simulink model "pokus07_video"  (R2023a)
settings: Solver=VariableStepAuto  StartTime=0.0  StopTime=10.0  RelTol=1e-3
undefined symbols (not defined in the file): c
libraries: Miscellaneous x840, Memory_Blocks_Lib x251, Decoders_Lib x10, simulink_extras x10, Counters_Lib x4, Bit_Multiplexers_Lib x1, Byte_Multiplexers_Lib x1
(part 2 of 5)

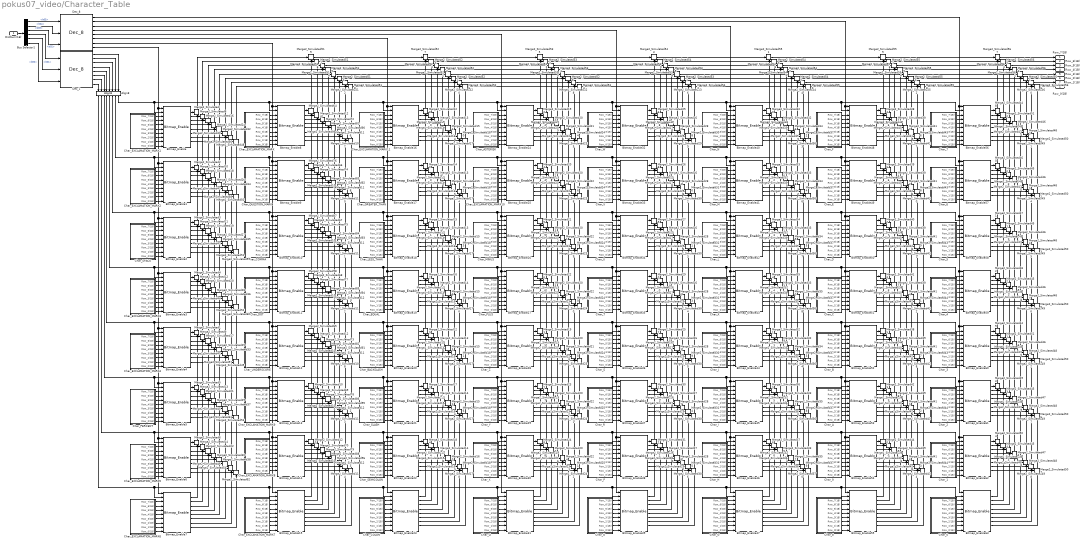
== system pokus07_video/Character_Table ==
  OrdNum(1B) : Inport
  Align8 : Miscellaneous/Align8  SystemSampleTime=-1  VariantActivationTime=update diagram  Latency=0  AutoFrameSizeCalculation=off
  Bitmap_Enable{,1..63} (64 alike) : Miscellaneous/Bitmap_Enable  SystemSampleTime=-1  VariantActivationTime=update diagram  Latency=0  AutoFrameSizeCalculation=off
  Bus Selector1 : BusSelector  OutputSignals=b05,b04,b03,b02,b01,b00
  Char_0 : Subsystem
  Char_1 : Subsystem
  Char_2 : Subsystem
  Char_3 : Subsystem
  Char_4 : Subsystem
  Char_5 : Subsystem
  Char_6 : Subsystem
  Char_7 : Subsystem
  Char_8 : Subsystem
  Char_9 : Subsystem
  Char_A : Subsystem
  Char_ASTERISK : Subsystem
  Char_B : Subsystem
  Char_BACKSLASH : Subsystem
  Char_C : Subsystem
  Char_COLON : Subsystem
  Char_COMMA : Subsystem
  Char_D : Subsystem
  Char_DOT : Subsystem
  Char_E : Subsystem
  Char_EQUAL : Subsystem
  Char_EXCLAMATION_MARK : Subsystem
  Char_EXCLAMATION_MARK1 : Subsystem
  Char_EXCLAMATION_MARK10 : Subsystem
  Char_EXCLAMATION_MARK11 : Subsystem
  Char_EXCLAMATION_MARK2 : Subsystem
  Char_EXCLAMATION_MARK3 : Subsystem
  Char_EXCLAMATION_MARK4 : Subsystem
  Char_EXCLAMATION_MARK5 : Subsystem
  Char_EXCLAMATION_MARK6 : Subsystem
  Char_EXCLAMATION_MARK7 : Subsystem
  Char_EXCLAMATION_MARK8 : Subsystem
  Char_EXCLAMATION_MARK9 : Subsystem
  Char_F : Subsystem
  Char_G : Subsystem
  Char_GREATER_THAN : Subsystem
  Char_H : Subsystem
  Char_I : Subsystem
  Char_J : Subsystem
  Char_K : Subsystem
  Char_L : Subsystem
  Char_LESS_THAN : Subsystem
  Char_M : Subsystem
  Char_MINUS : Subsystem
  Char_N : Subsystem
  Char_O : Subsystem
  Char_P : Subsystem
  Char_PERCENT : Subsystem
  Char_PLUS : Subsystem
  Char_Q : Subsystem
  Char_QUESTION_MARK : Subsystem
  Char_R : Subsystem
  Char_S : Subsystem
  Char_SEMICOLON : Subsystem
  Char_SLASH : Subsystem
  Char_SPACE : Subsystem
  Char_T : Subsystem
  Char_U : Subsystem
  Char_UNDERSCORE : Subsystem
  Char_V : Subsystem
  Char_W : Subsystem
  Char_X : Subsystem
  Char_Y : Subsystem
  Char_Z : Subsystem
  Dec_1 : Decoders_Lib/Dec_8  SystemSampleTime=-1  VariantActivationTime=update diagram  Latency=0  AutoFrameSizeCalculation=off
  Dec_8 : Decoders_Lib/Dec_8  SystemSampleTime=-1  VariantActivationTime=update diagram  Latency=0  AutoFrameSizeCalculation=off
  Merge2_Simulated{,1..6,8..14,16..22,24..30,32..38,40..46,48..54,56..62,64..70,72..79,81..88,90..96,98..105,107..114,116..123,126..134,136..143,145..152,154..160,162..169,171..178,180..187,190..198,200..207,209..216,218..224,226..233,235..242,244..251,254..262,264..271,273..280,282..288,290..297,299..306,308..315,318..326,328..335,337..344,346..352,354..361,363..370,372..379,382..390,392..399,401..408,410..416,418..425,427..434,436..443,446..454,456..463,465..472,474..480,482..489,491..498,500..507,510..567} (504 alike) : Miscellaneous/Merge2_Simulated  SystemSampleTime=-1  VariantActivationTime=update diagram  Latency=0  AutoFrameSizeCalculation=off
      settings: PortSchema="{\"entries\":[{\"content\":{\"sides\":[{\"content\":{\"connectorIds\":[\"In1\"]},\"type\":\"ConnectorPlacement.EquallySpacedRectSide\",\"uuid\":\"74758995-5ec8-49f8-a534-c3a678c5c312\"},{\"content\":{\"side\":\"RIGHT\"},\"type\":\"ConnectorPlacement.EquallySpacedRectSide\",\"uuid\":\"c467dbeb-9f00-48b9-a78d-a08162163a10\"},{\"content\":{\"connectorIds\":[\"Out1\"],\"side\":\"TOP\"},\"type\":\"ConnectorPlacement.EquallySpacedRectSide\",\"uuid\":\"39dea3b5-6733-4ade-ab22-e62d310be187\"},{\"content\":{\"connectorIds\":[\"In2\"],\"side\":\"BOTTOM\"},\"type\":\"ConnectorPlacement.EquallySpacedRectSide\",\"uuid\":\"73149fc1-24d9-4bdc-92e2-12fb1d742836\"}]},\"type\":\"ConnectorPlacement.EquallySpacedConnector\",\"uuid\":\"fd2226dc-a4d3-43ad-9cda-54babd09ac78\"}],\"packageUris\":[\"http://schema.mathworks.com/mf0/Connector/R2020b\"],\"version\":\"1.0\"}"
  Row_7(1B) : Outport
  Row_6(1B) : Outport  Port=2
  Row_5(1B) : Outport  Port=3
  Row_4(1B) : Outport  Port=4
  Row_3(1B) : Outport  Port=5
  Row_2(1B) : Outport  Port=6
  Row_1(1B) : Outport  Port=7
  Row_0(1B) : Outport  Port=8
  wires:
  Char_EXCLAMATION_MARK1/1(Row_7(1B)) -> Bitmap_Enable/3
  Char_EXCLAMATION_MARK1/2(Row_6(1B)) -> Bitmap_Enable/4
  Char_EXCLAMATION_MARK1/3(Row_5(1B)) -> Bitmap_Enable/5
  Char_EXCLAMATION_MARK1/4(Row_4(1B)) -> Bitmap_Enable/6
  Char_EXCLAMATION_MARK1/5(Row_3(1B)) -> Bitmap_Enable/7
  Char_EXCLAMATION_MARK1/6(Row_2(1B)) -> Bitmap_Enable/8
  Char_EXCLAMATION_MARK1/7(Row_1(1B)) -> Bitmap_Enable/9
  Char_EXCLAMATION_MARK1/8(Row_0(1B)) -> Bitmap_Enable/10
  Char_EXCLAMATION_MARK2/8(Row_0(1B)) -> Bitmap_Enable1/10
  Char_EXCLAMATION_MARK2/3(Row_5(1B)) -> Bitmap_Enable1/5
  Char_EXCLAMATION_MARK2/4(Row_4(1B)) -> Bitmap_Enable1/6
  Char_EXCLAMATION_MARK2/1(Row_7(1B)) -> Bitmap_Enable1/3
  Char_EXCLAMATION_MARK2/2(Row_6(1B)) -> Bitmap_Enable1/4
  Char_EXCLAMATION_MARK2/5(Row_3(1B)) -> Bitmap_Enable1/7
  Char_EXCLAMATION_MARK2/6(Row_2(1B)) -> Bitmap_Enable1/8
  Char_EXCLAMATION_MARK2/7(Row_1(1B)) -> Bitmap_Enable1/9
  Char_SPACE/8(Row_0(1B)) -> Bitmap_Enable2/10
  Char_SPACE/3(Row_5(1B)) -> Bitmap_Enable2/5
  Char_SPACE/4(Row_4(1B)) -> Bitmap_Enable2/6
  Char_SPACE/1(Row_7(1B)) -> Bitmap_Enable2/3
  Char_SPACE/2(Row_6(1B)) -> Bitmap_Enable2/4
  Char_SPACE/5(Row_3(1B)) -> Bitmap_Enable2/7
  Char_SPACE/6(Row_2(1B)) -> Bitmap_Enable2/8
  Char_SPACE/7(Row_1(1B)) -> Bitmap_Enable2/9
  Char_EXCLAMATION_MARK3/8(Row_0(1B)) -> Bitmap_Enable3/10
  Char_EXCLAMATION_MARK3/3(Row_5(1B)) -> Bitmap_Enable3/5
  Char_EXCLAMATION_MARK3/4(Row_4(1B)) -> Bitmap_Enable3/6
  Char_EXCLAMATION_MARK3/1(Row_7(1B)) -> Bitmap_Enable3/3
  Char_EXCLAMATION_MARK3/2(Row_6(1B)) -> Bitmap_Enable3/4
  Char_EXCLAMATION_MARK3/5(Row_3(1B)) -> Bitmap_Enable3/7
  Char_EXCLAMATION_MARK3/6(Row_2(1B)) -> Bitmap_Enable3/8
  Char_EXCLAMATION_MARK3/7(Row_1(1B)) -> Bitmap_Enable3/9
  Char_EXCLAMATION_MARK5/5(Row_3(1B)) -> Bitmap_Enable6/7
  Char_PERCENT/4(Row_4(1B)) -> Bitmap_Enable5/6
  Char_PERCENT/3(Row_5(1B)) -> Bitmap_Enable5/5
  Char_EXCLAMATION_MARK5/7(Row_1(1B)) -> Bitmap_Enable6/9
  Char_EXCLAMATION_MARK5/4(Row_4(1B)) -> Bitmap_Enable6/6
  Char_EXCLAMATION_MARK5/2(Row_6(1B)) -> Bitmap_Enable6/4
  Char_PERCENT/8(Row_0(1B)) -> Bitmap_Enable5/10
  Char_EXCLAMATION_MARK5/8(Row_0(1B)) -> Bitmap_Enable6/10
  Char_EXCLAMATION_MARK5/1(Row_7(1B)) -> Bitmap_Enable6/3
  Char_PERCENT/2(Row_6(1B)) -> Bitmap_Enable5/4
  Char_EXCLAMATION_MARK5/3(Row_5(1B)) -> Bitmap_Enable6/5
  Char_EXCLAMATION_MARK6/7(Row_1(1B)) -> Bitmap_Enable7/9
  Char_PERCENT/6(Row_2(1B)) -> Bitmap_Enable5/8
  Char_PERCENT/1(Row_7(1B)) -> Bitmap_Enable5/3
  Char_EXCLAMATION_MARK6/8(Row_0(1B)) -> Bitmap_Enable7/10
  Char_EXCLAMATION_MARK6/6(Row_2(1B)) -> Bitmap_Enable7/8
  Char_EXCLAMATION_MARK6/4(Row_4(1B)) -> Bitmap_Enable7/6
  Char_EXCLAMATION_MARK6/3(Row_5(1B)) -> Bitmap_Enable7/5
  Char_EXCLAMATION_MARK4/8(Row_0(1B)) -> Bitmap_Enable4/10
  Char_EXCLAMATION_MARK4/3(Row_5(1B)) -> Bitmap_Enable4/5
  Char_EXCLAMATION_MARK4/4(Row_4(1B)) -> Bitmap_Enable4/6
  Char_PERCENT/7(Row_1(1B)) -> Bitmap_Enable5/9
  Char_EXCLAMATION_MARK5/6(Row_2(1B)) -> Bitmap_Enable6/8
  Char_EXCLAMATION_MARK4/1(Row_7(1B)) -> Bitmap_Enable4/3
  Char_EXCLAMATION_MARK4/2(Row_6(1B)) -> Bitmap_Enable4/4
  Char_EXCLAMATION_MARK6/2(Row_6(1B)) -> Bitmap_Enable7/4
  Char_EXCLAMATION_MARK4/5(Row_3(1B)) -> Bitmap_Enable4/7
  Char_EXCLAMATION_MARK6/1(Row_7(1B)) -> Bitmap_Enable7/3
  Char_EXCLAMATION_MARK6/5(Row_3(1B)) -> Bitmap_Enable7/7
  Char_EXCLAMATION_MARK4/6(Row_2(1B)) -> Bitmap_Enable4/8
  Char_EXCLAMATION_MARK4/7(Row_1(1B)) -> Bitmap_Enable4/9
  Char_PERCENT/5(Row_3(1B)) -> Bitmap_Enable5/7
  Char_COMMA/5(Row_3(1B)) -> Bitmap_Enable10/7
  Char_QUESTION_MARK/4(Row_4(1B)) -> Bitmap_Enable9/6
  Char_QUESTION_MARK/3(Row_5(1B)) -> Bitmap_Enable9/5
  Char_COMMA/7(Row_1(1B)) -> Bitmap_Enable10/9
  Char_COMMA/4(Row_4(1B)) -> Bitmap_Enable10/6
  Char_COMMA/2(Row_6(1B)) -> Bitmap_Enable10/4
  Char_COMMA/1(Row_7(1B)) -> Bitmap_Enable10/3
  Char_QUESTION_MARK/2(Row_6(1B)) -> Bitmap_Enable9/4
  Char_COMMA/3(Row_5(1B)) -> Bitmap_Enable10/5
  Char_DOT/8(Row_0(1B)) -> Bitmap_Enable11/10
  Char_DOT/6(Row_2(1B)) -> Bitmap_Enable11/8
  Char_EXCLAMATION_MARK9/1(Row_7(1B)) -> Bitmap_Enable13/3
  Char_UNDERSCORE/1(Row_7(1B)) -> Bitmap_Enable12/3
  Char_EXCLAMATION_MARK9/2(Row_6(1B)) -> Bitmap_Enable13/4
  Char_EXCLAMATION_MARK8/3(Row_5(1B)) -> Bitmap_Enable14/4
  Char_EXCLAMATION_MARK9/4(Row_4(1B)) -> Bitmap_Enable13/6
  Char_EXCLAMATION_MARK8/8(Row_0(1B)) -> Bitmap_Enable14/9
  Char_EXCLAMATION_MARK8/7(Row_1(1B)) -> Bitmap_Enable14/8
  Char_EXCLAMATION_MARK8/5(Row_3(1B)) -> Bitmap_Enable14/6
  Char_EXCLAMATION_MARK7/8(Row_0(1B)) -> Bitmap_Enable15/10
  Char_UNDERSCORE/8(Row_0(1B)) -> Bitmap_Enable12/10
  Char_EXCLAMATION_MARK7/1(Row_7(1B)) -> Bitmap_Enable15/3
  Char_EXCLAMATION_MARK7/6(Row_2(1B)) -> Bitmap_Enable15/8
  Char_DOT/7(Row_1(1B)) -> Bitmap_Enable11/9
  Char_QUESTION_MARK/6(Row_2(1B)) -> Bitmap_Enable9/8
  Char_QUESTION_MARK/1(Row_7(1B)) -> Bitmap_Enable9/3
  Char_EXCLAMATION_MARK8/6(Row_2(1B)) -> Bitmap_Enable14/7
  Char_UNDERSCORE/5(Row_3(1B)) -> Bitmap_Enable12/7
  Char_EXCLAMATION_MARK9/5(Row_3(1B)) -> Bitmap_Enable13/7
  Char_UNDERSCORE/3(Row_5(1B)) -> Bitmap_Enable12/5
  Char_EXCLAMATION_MARK7/5(Row_3(1B)) -> Bitmap_Enable15/7
  ? -> Bitmap_Enable14/10
  Char_DOT/4(Row_4(1B)) -> Bitmap_Enable11/6
  Char_EXCLAMATION_MARK7/3(Row_5(1B)) -> Bitmap_Enable15/5
  Char_DOT/3(Row_5(1B)) -> Bitmap_Enable11/5
  Char_EXCLAMATION_MARK7/2(Row_6(1B)) -> Bitmap_Enable15/4
  Char_QUESTION_MARK/8(Row_0(1B)) -> Bitmap_Enable9/10
  Char_COMMA/8(Row_0(1B)) -> Bitmap_Enable10/10
  Char_EXCLAMATION_MARK7/4(Row_4(1B)) -> Bitmap_Enable15/6
  Char_UNDERSCORE/6(Row_2(1B)) -> Bitmap_Enable12/8
  Char_UNDERSCORE/7(Row_1(1B)) -> Bitmap_Enable12/9
  Char_UNDERSCORE/4(Row_4(1B)) -> Bitmap_Enable12/6
  Char_UNDERSCORE/2(Row_6(1B)) -> Bitmap_Enable12/4
  Char_EXCLAMATION_MARK8/2(Row_6(1B)) -> Bitmap_Enable14/3
  Char_EXCLAMATION_MARK9/8(Row_0(1B)) -> Bitmap_Enable13/10
  Char_EXCLAMATION_MARK9/6(Row_2(1B)) -> Bitmap_Enable13/8
  Char_EXCLAMATION_MARK9/7(Row_1(1B)) -> Bitmap_Enable13/9
  Char_EXCLAMATION_MARK9/3(Row_5(1B)) -> Bitmap_Enable13/5
  Char_EXCLAMATION_MARK/8(Row_0(1B)) -> Bitmap_Enable8/10
  Char_EXCLAMATION_MARK/3(Row_5(1B)) -> Bitmap_Enable8/5
  Char_EXCLAMATION_MARK7/7(Row_1(1B)) -> Bitmap_Enable15/9
  Char_EXCLAMATION_MARK/4(Row_4(1B)) -> Bitmap_Enable8/6
  Char_QUESTION_MARK/7(Row_1(1B)) -> Bitmap_Enable9/9
  Char_COMMA/6(Row_2(1B)) -> Bitmap_Enable10/8
  Char_EXCLAMATION_MARK/1(Row_7(1B)) -> Bitmap_Enable8/3
  Char_EXCLAMATION_MARK/2(Row_6(1B)) -> Bitmap_Enable8/4
  Char_DOT/2(Row_6(1B)) -> Bitmap_Enable11/4
  Char_EXCLAMATION_MARK/5(Row_3(1B)) -> Bitmap_Enable8/7
  Char_DOT/1(Row_7(1B)) -> Bitmap_Enable11/3
  Char_DOT/5(Row_3(1B)) -> Bitmap_Enable11/7
  Char_EXCLAMATION_MARK/6(Row_2(1B)) -> Bitmap_Enable8/8
  Char_EXCLAMATION_MARK/7(Row_1(1B)) -> Bitmap_Enable8/9
  Char_EXCLAMATION_MARK8/4(Row_4(1B)) -> Bitmap_Enable14/5
  Char_QUESTION_MARK/5(Row_3(1B)) -> Bitmap_Enable9/7
  Char_LESS_THAN/5(Row_3(1B)) -> Bitmap_Enable18/7
  Char_GREATER_THAN/4(Row_4(1B)) -> Bitmap_Enable17/6
  Char_GREATER_THAN/3(Row_5(1B)) -> Bitmap_Enable17/5
  Char_LESS_THAN/7(Row_1(1B)) -> Bitmap_Enable18/9
  Char_LESS_THAN/4(Row_4(1B)) -> Bitmap_Enable18/6
  Char_LESS_THAN/2(Row_6(1B)) -> Bitmap_Enable18/4
  Char_LESS_THAN/1(Row_7(1B)) -> Bitmap_Enable18/3
  Char_GREATER_THAN/2(Row_6(1B)) -> Bitmap_Enable17/4
  Char_LESS_THAN/3(Row_5(1B)) -> Bitmap_Enable18/5
  Char_EQUAL/8(Row_0(1B)) -> Bitmap_Enable19/10
  Char_EQUAL/6(Row_2(1B)) -> Bitmap_Enable19/8
  Char_SLASH/1(Row_7(1B)) -> Bitmap_Enable21/3
  Char_BACKSLASH/1(Row_7(1B)) -> Bitmap_Enable20/3
  Char_SLASH/2(Row_6(1B)) -> Bitmap_Enable21/4
  Char_SEMICOLON/2(Row_6(1B)) -> Bitmap_Enable22/4
  Char_SLASH/4(Row_4(1B)) -> Bitmap_Enable21/6
  Char_SEMICOLON/7(Row_1(1B)) -> Bitmap_Enable22/9
  Char_SEMICOLON/6(Row_2(1B)) -> Bitmap_Enable22/8
  Char_SEMICOLON/4(Row_4(1B)) -> Bitmap_Enable22/6
  Char_COLON/8(Row_0(1B)) -> Bitmap_Enable23/10
  Char_BACKSLASH/8(Row_0(1B)) -> Bitmap_Enable20/10
  Char_COLON/1(Row_7(1B)) -> Bitmap_Enable23/3
  Char_COLON/6(Row_2(1B)) -> Bitmap_Enable23/8
  Char_EQUAL/7(Row_1(1B)) -> Bitmap_Enable19/9
  Char_GREATER_THAN/6(Row_2(1B)) -> Bitmap_Enable17/8
  Char_GREATER_THAN/1(Row_7(1B)) -> Bitmap_Enable17/3
  Char_SEMICOLON/5(Row_3(1B)) -> Bitmap_Enable22/7
  Char_BACKSLASH/5(Row_3(1B)) -> Bitmap_Enable20/7
  Char_SLASH/5(Row_3(1B)) -> Bitmap_Enable21/7
  Char_BACKSLASH/3(Row_5(1B)) -> Bitmap_Enable20/5
  Char_COLON/5(Row_3(1B)) -> Bitmap_Enable23/7
  Char_SEMICOLON/8(Row_0(1B)) -> Bitmap_Enable22/10
  Char_EQUAL/4(Row_4(1B)) -> Bitmap_Enable19/6
  Char_COLON/3(Row_5(1B)) -> Bitmap_Enable23/5
  Char_EQUAL/3(Row_5(1B)) -> Bitmap_Enable19/5
  Char_COLON/2(Row_6(1B)) -> Bitmap_Enable23/4
  Char_GREATER_THAN/8(Row_0(1B)) -> Bitmap_Enable17/10
  Char_LESS_THAN/8(Row_0(1B)) -> Bitmap_Enable18/10
  Char_COLON/4(Row_4(1B)) -> Bitmap_Enable23/6
  Char_BACKSLASH/6(Row_2(1B)) -> Bitmap_Enable20/8
  Char_BACKSLASH/7(Row_1(1B)) -> Bitmap_Enable20/9
  Char_BACKSLASH/4(Row_4(1B)) -> Bitmap_Enable20/6
  Char_BACKSLASH/2(Row_6(1B)) -> Bitmap_Enable20/4
  Char_SEMICOLON/1(Row_7(1B)) -> Bitmap_Enable22/3
  Char_SLASH/8(Row_0(1B)) -> Bitmap_Enable21/10
  Char_SLASH/6(Row_2(1B)) -> Bitmap_Enable21/8
  Char_SLASH/7(Row_1(1B)) -> Bitmap_Enable21/9
  Char_SLASH/3(Row_5(1B)) -> Bitmap_Enable21/5
  Char_EXCLAMATION_MARK11/8(Row_0(1B)) -> Bitmap_Enable16/10
  Char_EXCLAMATION_MARK11/3(Row_5(1B)) -> Bitmap_Enable16/5
  Char_COLON/7(Row_1(1B)) -> Bitmap_Enable23/9
  Char_EXCLAMATION_MARK11/4(Row_4(1B)) -> Bitmap_Enable16/6
  Char_GREATER_THAN/7(Row_1(1B)) -> Bitmap_Enable17/9
  Char_LESS_THAN/6(Row_2(1B)) -> Bitmap_Enable18/8
  Char_EXCLAMATION_MARK11/1(Row_7(1B)) -> Bitmap_Enable16/3
  Char_EXCLAMATION_MARK11/2(Row_6(1B)) -> Bitmap_Enable16/4
  Char_EQUAL/2(Row_6(1B)) -> Bitmap_Enable19/4
  Char_EXCLAMATION_MARK11/5(Row_3(1B)) -> Bitmap_Enable16/7
  Char_EQUAL/1(Row_7(1B)) -> Bitmap_Enable19/3
  Char_EQUAL/5(Row_3(1B)) -> Bitmap_Enable19/7
  Char_EXCLAMATION_MARK11/6(Row_2(1B)) -> Bitmap_Enable16/8
  Char_EXCLAMATION_MARK11/7(Row_1(1B)) -> Bitmap_Enable16/9
  Char_SEMICOLON/3(Row_5(1B)) -> Bitmap_Enable22/5
  Char_GREATER_THAN/5(Row_3(1B)) -> Bitmap_Enable17/7
  Char_MINUS/5(Row_3(1B)) -> Bitmap_Enable26/7
  Char_EXCLAMATION_MARK10/4(Row_4(1B)) -> Bitmap_Enable25/6
  Char_EXCLAMATION_MARK10/3(Row_5(1B)) -> Bitmap_Enable25/5
  Char_MINUS/7(Row_1(1B)) -> Bitmap_Enable26/9
  Char_MINUS/4(Row_4(1B)) -> Bitmap_Enable26/6
  Char_MINUS/2(Row_6(1B)) -> Bitmap_Enable26/4
  Char_MINUS/1(Row_7(1B)) -> Bitmap_Enable26/3
  Char_EXCLAMATION_MARK10/2(Row_6(1B)) -> Bitmap_Enable25/4
  Char_MINUS/3(Row_5(1B)) -> Bitmap_Enable26/5
  Char_PLUS/8(Row_0(1B)) -> Bitmap_Enable27/10
  Char_PLUS/6(Row_2(1B)) -> Bitmap_Enable27/8
  Char_Y/1(Row_7(1B)) -> Bitmap_Enable29/3
  Char_Z/1(Row_7(1B)) -> Bitmap_Enable28/3
  Char_Y/2(Row_6(1B)) -> Bitmap_Enable29/4
  Char_X/2(Row_6(1B)) -> Bitmap_Enable30/4
  Char_Y/4(Row_4(1B)) -> Bitmap_Enable29/6
  Char_X/7(Row_1(1B)) -> Bitmap_Enable30/9
  Char_X/6(Row_2(1B)) -> Bitmap_Enable30/8
  Char_X/4(Row_4(1B)) -> Bitmap_Enable30/6
  Char_Q/8(Row_0(1B)) -> Bitmap_Enable31/10
  Char_Z/8(Row_0(1B)) -> Bitmap_Enable28/10
  Char_Q/1(Row_7(1B)) -> Bitmap_Enable31/3
  Char_Q/6(Row_2(1B)) -> Bitmap_Enable31/8
  Char_PLUS/7(Row_1(1B)) -> Bitmap_Enable27/9
  Char_EXCLAMATION_MARK10/6(Row_2(1B)) -> Bitmap_Enable25/8
  Char_EXCLAMATION_MARK10/1(Row_7(1B)) -> Bitmap_Enable25/3
  Char_X/5(Row_3(1B)) -> Bitmap_Enable30/7
  Char_Z/5(Row_3(1B)) -> Bitmap_Enable28/7
  Char_Y/5(Row_3(1B)) -> Bitmap_Enable29/7
  Char_Z/3(Row_5(1B)) -> Bitmap_Enable28/5
  Char_Q/5(Row_3(1B)) -> Bitmap_Enable31/7
  Char_X/8(Row_0(1B)) -> Bitmap_Enable30/10
  Char_PLUS/4(Row_4(1B)) -> Bitmap_Enable27/6
  Char_Q/3(Row_5(1B)) -> Bitmap_Enable31/5
  Char_PLUS/3(Row_5(1B)) -> Bitmap_Enable27/5
  Char_Q/2(Row_6(1B)) -> Bitmap_Enable31/4
  Char_EXCLAMATION_MARK10/8(Row_0(1B)) -> Bitmap_Enable25/10
  Char_MINUS/8(Row_0(1B)) -> Bitmap_Enable26/10
  Char_Q/4(Row_4(1B)) -> Bitmap_Enable31/6
  Char_Z/6(Row_2(1B)) -> Bitmap_Enable28/8
  Char_Z/7(Row_1(1B)) -> Bitmap_Enable28/9
  Char_Z/4(Row_4(1B)) -> Bitmap_Enable28/6
  Char_Z/2(Row_6(1B)) -> Bitmap_Enable28/4
  Char_X/1(Row_7(1B)) -> Bitmap_Enable30/3
  Char_Y/8(Row_0(1B)) -> Bitmap_Enable29/10
  Char_Y/6(Row_2(1B)) -> Bitmap_Enable29/8
  Char_Y/7(Row_1(1B)) -> Bitmap_Enable29/9
  Char_Y/3(Row_5(1B)) -> Bitmap_Enable29/5
  Char_ASTERISK/8(Row_0(1B)) -> Bitmap_Enable24/10
  Char_ASTERISK/3(Row_5(1B)) -> Bitmap_Enable24/5
  Char_Q/7(Row_1(1B)) -> Bitmap_Enable31/9
  Char_ASTERISK/4(Row_4(1B)) -> Bitmap_Enable24/6
  Char_EXCLAMATION_MARK10/7(Row_1(1B)) -> Bitmap_Enable25/9
  Char_MINUS/6(Row_2(1B)) -> Bitmap_Enable26/8
  Char_ASTERISK/1(Row_7(1B)) -> Bitmap_Enable24/3
  Char_ASTERISK/2(Row_6(1B)) -> Bitmap_Enable24/4
  Char_PLUS/2(Row_6(1B)) -> Bitmap_Enable27/4
  Char_ASTERISK/5(Row_3(1B)) -> Bitmap_Enable24/7
  Char_PLUS/1(Row_7(1B)) -> Bitmap_Enable27/3
  Char_PLUS/5(Row_3(1B)) -> Bitmap_Enable27/7
  Char_ASTERISK/6(Row_2(1B)) -> Bitmap_Enable24/8
  Char_ASTERISK/7(Row_1(1B)) -> Bitmap_Enable24/9
  Char_X/3(Row_5(1B)) -> Bitmap_Enable30/5
  Char_EXCLAMATION_MARK10/5(Row_3(1B)) -> Bitmap_Enable25/7
  Char_U/5(Row_3(1B)) -> Bitmap_Enable34/7
  Char_V/4(Row_4(1B)) -> Bitmap_Enable33/6
  Char_V/3(Row_5(1B)) -> Bitmap_Enable33/5
  Char_U/7(Row_1(1B)) -> Bitmap_Enable34/9
  Char_U/4(Row_4(1B)) -> Bitmap_Enable34/6
  Char_U/2(Row_6(1B)) -> Bitmap_Enable34/4
  Char_U/1(Row_7(1B)) -> Bitmap_Enable34/3
  Char_V/2(Row_6(1B)) -> Bitmap_Enable33/4
  Char_U/3(Row_5(1B)) -> Bitmap_Enable34/5
  Char_T/8(Row_0(1B)) -> Bitmap_Enable35/10
  Char_T/6(Row_2(1B)) -> Bitmap_Enable35/8
  Char_R/1(Row_7(1B)) -> Bitmap_Enable37/3
  Char_S/1(Row_7(1B)) -> Bitmap_Enable36/3
  Char_R/2(Row_6(1B)) -> Bitmap_Enable37/4
  Char_P/2(Row_6(1B)) -> Bitmap_Enable38/4
  Char_R/4(Row_4(1B)) -> Bitmap_Enable37/6
  Char_P/7(Row_1(1B)) -> Bitmap_Enable38/9
  Char_P/6(Row_2(1B)) -> Bitmap_Enable38/8
  Char_P/4(Row_4(1B)) -> Bitmap_Enable38/6
  Char_O/8(Row_0(1B)) -> Bitmap_Enable39/10
  Char_S/8(Row_0(1B)) -> Bitmap_Enable36/10
  Char_O/1(Row_7(1B)) -> Bitmap_Enable39/3
  Char_O/6(Row_2(1B)) -> Bitmap_Enable39/8
  Char_T/7(Row_1(1B)) -> Bitmap_Enable35/9
  Char_V/6(Row_2(1B)) -> Bitmap_Enable33/8
  Char_V/1(Row_7(1B)) -> Bitmap_Enable33/3
  Char_P/5(Row_3(1B)) -> Bitmap_Enable38/7
  Char_S/5(Row_3(1B)) -> Bitmap_Enable36/7
  Char_R/5(Row_3(1B)) -> Bitmap_Enable37/7
  Char_S/3(Row_5(1B)) -> Bitmap_Enable36/5
  Char_O/5(Row_3(1B)) -> Bitmap_Enable39/7
  Char_P/8(Row_0(1B)) -> Bitmap_Enable38/10
  Char_T/4(Row_4(1B)) -> Bitmap_Enable35/6
  Char_O/3(Row_5(1B)) -> Bitmap_Enable39/5
  Char_T/3(Row_5(1B)) -> Bitmap_Enable35/5
  Char_O/2(Row_6(1B)) -> Bitmap_Enable39/4
  Char_V/8(Row_0(1B)) -> Bitmap_Enable33/10
  Char_U/8(Row_0(1B)) -> Bitmap_Enable34/10
  Char_O/4(Row_4(1B)) -> Bitmap_Enable39/6
  Char_S/6(Row_2(1B)) -> Bitmap_Enable36/8
  Char_S/7(Row_1(1B)) -> Bitmap_Enable36/9
  Char_S/4(Row_4(1B)) -> Bitmap_Enable36/6
  Char_S/2(Row_6(1B)) -> Bitmap_Enable36/4
  Char_P/1(Row_7(1B)) -> Bitmap_Enable38/3
  Char_R/8(Row_0(1B)) -> Bitmap_Enable37/10
  Char_R/6(Row_2(1B)) -> Bitmap_Enable37/8
  Char_R/7(Row_1(1B)) -> Bitmap_Enable37/9
  Char_R/3(Row_5(1B)) -> Bitmap_Enable37/5
  Char_W/8(Row_0(1B)) -> Bitmap_Enable32/10
  Char_W/3(Row_5(1B)) -> Bitmap_Enable32/5
  Char_O/7(Row_1(1B)) -> Bitmap_Enable39/9
  Char_W/4(Row_4(1B)) -> Bitmap_Enable32/6
  Char_V/7(Row_1(1B)) -> Bitmap_Enable33/9
  Char_U/6(Row_2(1B)) -> Bitmap_Enable34/8
  Char_W/1(Row_7(1B)) -> Bitmap_Enable32/3
  Char_W/2(Row_6(1B)) -> Bitmap_Enable32/4
  Char_T/2(Row_6(1B)) -> Bitmap_Enable35/4
  Char_W/5(Row_3(1B)) -> Bitmap_Enable32/7
  Char_T/1(Row_7(1B)) -> Bitmap_Enable35/3
  Char_T/5(Row_3(1B)) -> Bitmap_Enable35/7
  Char_W/6(Row_2(1B)) -> Bitmap_Enable32/8
  Char_W/7(Row_1(1B)) -> Bitmap_Enable32/9
  Char_P/3(Row_5(1B)) -> Bitmap_Enable38/5
  Char_V/5(Row_3(1B)) -> Bitmap_Enable33/7
  Char_L/5(Row_3(1B)) -> Bitmap_Enable42/7
  Char_M/4(Row_4(1B)) -> Bitmap_Enable41/6
  Char_M/3(Row_5(1B)) -> Bitmap_Enable41/5
  Char_L/7(Row_1(1B)) -> Bitmap_Enable42/9
  Char_L/4(Row_4(1B)) -> Bitmap_Enable42/6
  Char_L/2(Row_6(1B)) -> Bitmap_Enable42/4
  Char_L/1(Row_7(1B)) -> Bitmap_Enable42/3
  Char_M/2(Row_6(1B)) -> Bitmap_Enable41/4
  Char_L/3(Row_5(1B)) -> Bitmap_Enable42/5
  Char_K/8(Row_0(1B)) -> Bitmap_Enable43/10
  Char_K/6(Row_2(1B)) -> Bitmap_Enable43/8
  Char_I/1(Row_7(1B)) -> Bitmap_Enable45/3
  Char_J/1(Row_7(1B)) -> Bitmap_Enable44/3
  Char_I/2(Row_6(1B)) -> Bitmap_Enable45/4
  Char_H/2(Row_6(1B)) -> Bitmap_Enable46/4
  Char_I/4(Row_4(1B)) -> Bitmap_Enable45/6
  Char_H/7(Row_1(1B)) -> Bitmap_Enable46/9
  Char_H/6(Row_2(1B)) -> Bitmap_Enable46/8
  Char_H/4(Row_4(1B)) -> Bitmap_Enable46/6
  Char_G/8(Row_0(1B)) -> Bitmap_Enable47/10
  Char_J/8(Row_0(1B)) -> Bitmap_Enable44/10
  Char_G/1(Row_7(1B)) -> Bitmap_Enable47/3
  Char_G/6(Row_2(1B)) -> Bitmap_Enable47/8
  Char_K/7(Row_1(1B)) -> Bitmap_Enable43/9
  Char_M/6(Row_2(1B)) -> Bitmap_Enable41/8
  Char_M/1(Row_7(1B)) -> Bitmap_Enable41/3
  Char_H/5(Row_3(1B)) -> Bitmap_Enable46/7
  Char_J/5(Row_3(1B)) -> Bitmap_Enable44/7
  Char_I/5(Row_3(1B)) -> Bitmap_Enable45/7
  Char_J/3(Row_5(1B)) -> Bitmap_Enable44/5
  Char_G/5(Row_3(1B)) -> Bitmap_Enable47/7
  Char_H/8(Row_0(1B)) -> Bitmap_Enable46/10
  Char_K/4(Row_4(1B)) -> Bitmap_Enable43/6
  Char_G/3(Row_5(1B)) -> Bitmap_Enable47/5
  Char_K/3(Row_5(1B)) -> Bitmap_Enable43/5
  Char_G/2(Row_6(1B)) -> Bitmap_Enable47/4
  Char_M/8(Row_0(1B)) -> Bitmap_Enable41/10
  Char_L/8(Row_0(1B)) -> Bitmap_Enable42/10
  Char_G/4(Row_4(1B)) -> Bitmap_Enable47/6
  Char_J/6(Row_2(1B)) -> Bitmap_Enable44/8
  Char_J/7(Row_1(1B)) -> Bitmap_Enable44/9
  Char_J/4(Row_4(1B)) -> Bitmap_Enable44/6
  Char_J/2(Row_6(1B)) -> Bitmap_Enable44/4
  Char_H/1(Row_7(1B)) -> Bitmap_Enable46/3
  Char_I/8(Row_0(1B)) -> Bitmap_Enable45/10
  Char_I/6(Row_2(1B)) -> Bitmap_Enable45/8
  Char_I/7(Row_1(1B)) -> Bitmap_Enable45/9
  Char_I/3(Row_5(1B)) -> Bitmap_Enable45/5
  Char_N/8(Row_0(1B)) -> Bitmap_Enable40/10
  Char_N/3(Row_5(1B)) -> Bitmap_Enable40/5
  Char_G/7(Row_1(1B)) -> Bitmap_Enable47/9
  Char_N/4(Row_4(1B)) -> Bitmap_Enable40/6
  Char_M/7(Row_1(1B)) -> Bitmap_Enable41/9
  Char_L/6(Row_2(1B)) -> Bitmap_Enable42/8
  Char_N/1(Row_7(1B)) -> Bitmap_Enable40/3
  Char_N/2(Row_6(1B)) -> Bitmap_Enable40/4
  Char_K/2(Row_6(1B)) -> Bitmap_Enable43/4
  Char_N/5(Row_3(1B)) -> Bitmap_Enable40/7
  Char_K/1(Row_7(1B)) -> Bitmap_Enable43/3
  Char_K/5(Row_3(1B)) -> Bitmap_Enable43/7
  Char_N/6(Row_2(1B)) -> Bitmap_Enable40/8
  Char_N/7(Row_1(1B)) -> Bitmap_Enable40/9
  Char_H/3(Row_5(1B)) -> Bitmap_Enable46/5
  Char_M/5(Row_3(1B)) -> Bitmap_Enable41/7
  Char_D/5(Row_3(1B)) -> Bitmap_Enable50/7
  Char_E/4(Row_4(1B)) -> Bitmap_Enable49/6
  Char_E/3(Row_5(1B)) -> Bitmap_Enable49/5
  Char_D/7(Row_1(1B)) -> Bitmap_Enable50/9
  Char_D/4(Row_4(1B)) -> Bitmap_Enable50/6
  Char_D/2(Row_6(1B)) -> Bitmap_Enable50/4
  Char_D/1(Row_7(1B)) -> Bitmap_Enable50/3
  Char_E/2(Row_6(1B)) -> Bitmap_Enable49/4
  Char_D/3(Row_5(1B)) -> Bitmap_Enable50/5
  Char_C/8(Row_0(1B)) -> Bitmap_Enable51/10
  Char_C/6(Row_2(1B)) -> Bitmap_Enable51/8
  Char_A/1(Row_7(1B)) -> Bitmap_Enable53/3
  Char_B/1(Row_7(1B)) -> Bitmap_Enable52/3
  Char_A/2(Row_6(1B)) -> Bitmap_Enable53/4
  Char_9/2(Row_6(1B)) -> Bitmap_Enable54/4
  Char_A/4(Row_4(1B)) -> Bitmap_Enable53/6
  Char_9/7(Row_1(1B)) -> Bitmap_Enable54/9
  Char_9/6(Row_2(1B)) -> Bitmap_Enable54/8
  Char_9/4(Row_4(1B)) -> Bitmap_Enable54/6
  Char_8/8(Row_0(1B)) -> Bitmap_Enable55/10
  Char_B/8(Row_0(1B)) -> Bitmap_Enable52/10
  Char_8/1(Row_7(1B)) -> Bitmap_Enable55/3
  Char_8/6(Row_2(1B)) -> Bitmap_Enable55/8
  Char_C/7(Row_1(1B)) -> Bitmap_Enable51/9
  Char_E/6(Row_2(1B)) -> Bitmap_Enable49/8
  Char_E/1(Row_7(1B)) -> Bitmap_Enable49/3
  Char_9/5(Row_3(1B)) -> Bitmap_Enable54/7
  Char_B/5(Row_3(1B)) -> Bitmap_Enable52/7
  Char_A/5(Row_3(1B)) -> Bitmap_Enable53/7
  Char_B/3(Row_5(1B)) -> Bitmap_Enable52/5
  Char_8/5(Row_3(1B)) -> Bitmap_Enable55/7
  Char_9/8(Row_0(1B)) -> Bitmap_Enable54/10
  Char_C/4(Row_4(1B)) -> Bitmap_Enable51/6
  Char_8/3(Row_5(1B)) -> Bitmap_Enable55/5
  Char_C/3(Row_5(1B)) -> Bitmap_Enable51/5
  Char_8/2(Row_6(1B)) -> Bitmap_Enable55/4
  Char_E/8(Row_0(1B)) -> Bitmap_Enable49/10
  Char_D/8(Row_0(1B)) -> Bitmap_Enable50/10
  Char_8/4(Row_4(1B)) -> Bitmap_Enable55/6
  Char_B/6(Row_2(1B)) -> Bitmap_Enable52/8
  Char_B/7(Row_1(1B)) -> Bitmap_Enable52/9
  Char_B/4(Row_4(1B)) -> Bitmap_Enable52/6
  Char_B/2(Row_6(1B)) -> Bitmap_Enable52/4
  Char_9/1(Row_7(1B)) -> Bitmap_Enable54/3
  Char_A/8(Row_0(1B)) -> Bitmap_Enable53/10
  Char_A/6(Row_2(1B)) -> Bitmap_Enable53/8
  Char_A/7(Row_1(1B)) -> Bitmap_Enable53/9
  Char_A/3(Row_5(1B)) -> Bitmap_Enable53/5
  Char_F/8(Row_0(1B)) -> Bitmap_Enable48/10
  Char_F/3(Row_5(1B)) -> Bitmap_Enable48/5
  Char_8/7(Row_1(1B)) -> Bitmap_Enable55/9
  Char_F/4(Row_4(1B)) -> Bitmap_Enable48/6
  Char_E/7(Row_1(1B)) -> Bitmap_Enable49/9
  Char_D/6(Row_2(1B)) -> Bitmap_Enable50/8
  Char_F/1(Row_7(1B)) -> Bitmap_Enable48/3
  Char_F/2(Row_6(1B)) -> Bitmap_Enable48/4
  Char_C/2(Row_6(1B)) -> Bitmap_Enable51/4
  Char_F/5(Row_3(1B)) -> Bitmap_Enable48/7
  Char_C/1(Row_7(1B)) -> Bitmap_Enable51/3
  Char_C/5(Row_3(1B)) -> Bitmap_Enable51/7
  Char_F/6(Row_2(1B)) -> Bitmap_Enable48/8
  Char_F/7(Row_1(1B)) -> Bitmap_Enable48/9
  Char_9/3(Row_5(1B)) -> Bitmap_Enable54/5
  Char_E/5(Row_3(1B)) -> Bitmap_Enable49/7
  Char_5/5(Row_3(1B)) -> Bitmap_Enable58/7
  Char_6/4(Row_4(1B)) -> Bitmap_Enable57/6
  Char_6/3(Row_5(1B)) -> Bitmap_Enable57/5
  Char_5/7(Row_1(1B)) -> Bitmap_Enable58/9
  Char_5/4(Row_4(1B)) -> Bitmap_Enable58/6
  Char_5/2(Row_6(1B)) -> Bitmap_Enable58/4
  Char_5/1(Row_7(1B)) -> Bitmap_Enable58/3
  Char_6/2(Row_6(1B)) -> Bitmap_Enable57/4
  Char_5/3(Row_5(1B)) -> Bitmap_Enable58/5
  Char_4/8(Row_0(1B)) -> Bitmap_Enable59/10
  Char_4/6(Row_2(1B)) -> Bitmap_Enable59/8
  Char_2/1(Row_7(1B)) -> Bitmap_Enable61/3
  Char_3/1(Row_7(1B)) -> Bitmap_Enable60/3
  Char_2/2(Row_6(1B)) -> Bitmap_Enable61/4
  Char_1/2(Row_6(1B)) -> Bitmap_Enable62/4
  Char_2/4(Row_4(1B)) -> Bitmap_Enable61/6
  Char_1/7(Row_1(1B)) -> Bitmap_Enable62/9
  Char_1/6(Row_2(1B)) -> Bitmap_Enable62/8
  Char_1/4(Row_4(1B)) -> Bitmap_Enable62/6
  Char_0/8(Row_0(1B)) -> Bitmap_Enable63/10
  Char_3/8(Row_0(1B)) -> Bitmap_Enable60/10
  Char_0/1(Row_7(1B)) -> Bitmap_Enable63/3
  Char_0/6(Row_2(1B)) -> Bitmap_Enable63/8
  Char_4/7(Row_1(1B)) -> Bitmap_Enable59/9
  Char_6/6(Row_2(1B)) -> Bitmap_Enable57/8
  Char_6/1(Row_7(1B)) -> Bitmap_Enable57/3
  Char_1/5(Row_3(1B)) -> Bitmap_Enable62/7
  Char_3/5(Row_3(1B)) -> Bitmap_Enable60/7
  Char_2/5(Row_3(1B)) -> Bitmap_Enable61/7
  Char_3/3(Row_5(1B)) -> Bitmap_Enable60/5
  Char_0/5(Row_3(1B)) -> Bitmap_Enable63/7
  Char_1/8(Row_0(1B)) -> Bitmap_Enable62/10
  Char_4/4(Row_4(1B)) -> Bitmap_Enable59/6
  Char_0/3(Row_5(1B)) -> Bitmap_Enable63/5
  Char_4/3(Row_5(1B)) -> Bitmap_Enable59/5
  Char_0/2(Row_6(1B)) -> Bitmap_Enable63/4
  Char_6/8(Row_0(1B)) -> Bitmap_Enable57/10
  Char_5/8(Row_0(1B)) -> Bitmap_Enable58/10
  Char_0/4(Row_4(1B)) -> Bitmap_Enable63/6
  Char_3/6(Row_2(1B)) -> Bitmap_Enable60/8
  Char_3/7(Row_1(1B)) -> Bitmap_Enable60/9
  Char_3/4(Row_4(1B)) -> Bitmap_Enable60/6
  Char_3/2(Row_6(1B)) -> Bitmap_Enable60/4
  Char_1/1(Row_7(1B)) -> Bitmap_Enable62/3
  Char_2/8(Row_0(1B)) -> Bitmap_Enable61/10
  Char_2/6(Row_2(1B)) -> Bitmap_Enable61/8
  Char_2/7(Row_1(1B)) -> Bitmap_Enable61/9
  Char_2/3(Row_5(1B)) -> Bitmap_Enable61/5
  Char_7/8(Row_0(1B)) -> Bitmap_Enable56/10
  Char_7/3(Row_5(1B)) -> Bitmap_Enable56/5
  Char_0/7(Row_1(1B)) -> Bitmap_Enable63/9
  Char_7/4(Row_4(1B)) -> Bitmap_Enable56/6
  Char_6/7(Row_1(1B)) -> Bitmap_Enable57/9
  Char_5/6(Row_2(1B)) -> Bitmap_Enable58/8
  Char_7/1(Row_7(1B)) -> Bitmap_Enable56/3
  Char_7/2(Row_6(1B)) -> Bitmap_Enable56/4
  Char_4/2(Row_6(1B)) -> Bitmap_Enable59/4
  Char_7/5(Row_3(1B)) -> Bitmap_Enable56/7
  Char_4/1(Row_7(1B)) -> Bitmap_Enable59/3
  Char_4/5(Row_3(1B)) -> Bitmap_Enable59/7
  Char_7/6(Row_2(1B)) -> Bitmap_Enable56/8
  Char_7/7(Row_1(1B)) -> Bitmap_Enable56/9
  Char_1/3(Row_5(1B)) -> Bitmap_Enable62/5
  Char_6/5(Row_3(1B)) -> Bitmap_Enable57/7
  Bitmap_Enable/1 -> Merge2_Simulated/1
  Merge2_Simulated2/1 -> Merge2_Simulated/2
  Bitmap_Enable1/1 -> Merge2_Simulated2/1
  Bitmap_Enable2/1 -> Merge2_Simulated3/1
  Merge2_Simulated3/1 -> Merge2_Simulated2/2
  Merge2_Simulated4/1 -> Merge2_Simulated3/2
  Bitmap_Enable3/1 -> Merge2_Simulated4/1
  Merge2_Simulated5/1 -> Merge2_Simulated1/2
  Bitmap_Enable4/1 -> Merge2_Simulated1/1
  Bitmap_Enable6/1 -> Merge2_Simulated6/1
  Bitmap_Enable5/1 -> Merge2_Simulated5/1
  Bitmap_Enable7/1 -> Merge2_Simulated6/2
  Merge2_Simulated6/1 -> Merge2_Simulated5/2
  Merge2_Simulated1/1 -> Merge2_Simulated4/2
  Merge2_Simulated10/1 -> Merge2_Simulated8/2
  Bitmap_Enable7/2 -> Merge2_Simulated14/2
  Merge2_Simulated13/1 -> Merge2_Simulated9/2
  Merge2_Simulated14/1 -> Merge2_Simulated13/2
  Merge2_Simulated12/1 -> Merge2_Simulated11/2
  Merge2_Simulated11/1 -> Merge2_Simulated10/2
  Merge2_Simulated9/1 -> Merge2_Simulated12/2
  Merge2_Simulated18/1 -> Merge2_Simulated16/2
  Bitmap_Enable7/3 -> Merge2_Simulated22/2
  Merge2_Simulated21/1 -> Merge2_Simulated17/2
  Merge2_Simulated22/1 -> Merge2_Simulated21/2
  Merge2_Simulated20/1 -> Merge2_Simulated19/2
  Merge2_Simulated19/1 -> Merge2_Simulated18/2
  Merge2_Simulated17/1 -> Merge2_Simulated20/2
  Merge2_Simulated26/1 -> Merge2_Simulated24/2
  Bitmap_Enable7/4 -> Merge2_Simulated30/2
  Merge2_Simulated29/1 -> Merge2_Simulated25/2
  Merge2_Simulated30/1 -> Merge2_Simulated29/2
  Merge2_Simulated28/1 -> Merge2_Simulated27/2
  Merge2_Simulated27/1 -> Merge2_Simulated26/2
  Merge2_Simulated25/1 -> Merge2_Simulated28/2
  Merge2_Simulated34/1 -> Merge2_Simulated32/2
  Bitmap_Enable7/5 -> Merge2_Simulated38/2
  Merge2_Simulated37/1 -> Merge2_Simulated33/2
  Merge2_Simulated38/1 -> Merge2_Simulated37/2
  Merge2_Simulated36/1 -> Merge2_Simulated35/2
  Merge2_Simulated35/1 -> Merge2_Simulated34/2
  Merge2_Simulated33/1 -> Merge2_Simulated36/2
  Merge2_Simulated42/1 -> Merge2_Simulated40/2
  Bitmap_Enable7/6 -> Merge2_Simulated46/2
  Merge2_Simulated45/1 -> Merge2_Simulated41/2
  Merge2_Simulated46/1 -> Merge2_Simulated45/2
  Merge2_Simulated44/1 -> Merge2_Simulated43/2
  Merge2_Simulated43/1 -> Merge2_Simulated42/2
  Merge2_Simulated41/1 -> Merge2_Simulated44/2
  Merge2_Simulated50/1 -> Merge2_Simulated48/2
  Bitmap_Enable7/7 -> Merge2_Simulated54/2
  Merge2_Simulated53/1 -> Merge2_Simulated49/2
  Merge2_Simulated54/1 -> Merge2_Simulated53/2
  Merge2_Simulated52/1 -> Merge2_Simulated51/2
  Merge2_Simulated51/1 -> Merge2_Simulated50/2
  Merge2_Simulated49/1 -> Merge2_Simulated52/2
  Merge2_Simulated58/1 -> Merge2_Simulated56/2
  Bitmap_Enable7/8 -> Merge2_Simulated62/2
  Merge2_Simulated61/1 -> Merge2_Simulated57/2
  Merge2_Simulated62/1 -> Merge2_Simulated61/2
  Merge2_Simulated60/1 -> Merge2_Simulated59/2
  Merge2_Simulated59/1 -> Merge2_Simulated58/2
  Merge2_Simulated57/1 -> Merge2_Simulated60/2
  Bitmap_Enable/2 -> Merge2_Simulated8/1
  Bitmap_Enable/3 -> Merge2_Simulated16/1
  Bitmap_Enable/4 -> Merge2_Simulated24/1
  Bitmap_Enable/5 -> Merge2_Simulated32/1
  Bitmap_Enable/6 -> Merge2_Simulated40/1
  Bitmap_Enable/7 -> Merge2_Simulated48/1
  Bitmap_Enable/8 -> Merge2_Simulated56/1
  Bitmap_Enable1/2 -> Merge2_Simulated10/1
  Bitmap_Enable1/3 -> Merge2_Simulated18/1
  Bitmap_Enable1/4 -> Merge2_Simulated26/1
  Bitmap_Enable1/5 -> Merge2_Simulated34/1
  Bitmap_Enable1/6 -> Merge2_Simulated42/1
  Bitmap_Enable1/7 -> Merge2_Simulated50/1
  Bitmap_Enable1/8 -> Merge2_Simulated58/1
  Bitmap_Enable2/2 -> Merge2_Simulated11/1
  Bitmap_Enable2/3 -> Merge2_Simulated19/1
  Bitmap_Enable2/4 -> Merge2_Simulated27/1
  Bitmap_Enable2/5 -> Merge2_Simulated35/1
  Bitmap_Enable2/6 -> Merge2_Simulated43/1
  Bitmap_Enable2/7 -> Merge2_Simulated51/1
  Bitmap_Enable2/8 -> Merge2_Simulated59/1
  Bitmap_Enable3/2 -> Merge2_Simulated12/1
  Bitmap_Enable3/3 -> Merge2_Simulated20/1
  Bitmap_Enable3/4 -> Merge2_Simulated28/1
  Bitmap_Enable3/5 -> Merge2_Simulated36/1
  Bitmap_Enable3/6 -> Merge2_Simulated44/1
  Bitmap_Enable3/7 -> Merge2_Simulated52/1
  Bitmap_Enable3/8 -> Merge2_Simulated60/1
  Bitmap_Enable4/2 -> Merge2_Simulated9/1
  Bitmap_Enable4/3 -> Merge2_Simulated17/1
  Bitmap_Enable4/4 -> Merge2_Simulated25/1
  Bitmap_Enable4/5 -> Merge2_Simulated33/1
  Bitmap_Enable4/6 -> Merge2_Simulated41/1
  Bitmap_Enable4/7 -> Merge2_Simulated49/1
  Bitmap_Enable4/8 -> Merge2_Simulated57/1
  Bitmap_Enable5/2 -> Merge2_Simulated13/1
  Bitmap_Enable5/3 -> Merge2_Simulated21/1
  Bitmap_Enable5/4 -> Merge2_Simulated29/1
  Bitmap_Enable5/5 -> Merge2_Simulated37/1
  Bitmap_Enable5/6 -> Merge2_Simulated45/1
  Bitmap_Enable5/7 -> Merge2_Simulated53/1
  Bitmap_Enable5/8 -> Merge2_Simulated61/1
  Bitmap_Enable6/2 -> Merge2_Simulated14/1
  Bitmap_Enable6/3 -> Merge2_Simulated22/1
  Bitmap_Enable6/4 -> Merge2_Simulated30/1
  Bitmap_Enable6/5 -> Merge2_Simulated38/1
  Bitmap_Enable6/6 -> Merge2_Simulated46/1
  Bitmap_Enable6/7 -> Merge2_Simulated54/1
  Bitmap_Enable6/8 -> Merge2_Simulated62/1
  Merge2_Simulated70/1 -> Merge2_Simulated69/2
  Bitmap_Enable15/2 -> Merge2_Simulated70/2
  Merge2_Simulated69/1 -> Merge2_Simulated127/2
  Merge2_Simulated68/1 -> Merge2_Simulated67/2
  Bitmap_Enable14/6 -> Merge2_Simulated105/1
  Merge2_Simulated77/1 -> Merge2_Simulated75/2
  Merge2_Simulated75/1 -> Merge2_Simulated74/2
  Merge2_Simulated79/1 -> Merge2_Simulated78/2
  Bitmap_Enable15/3 -> Merge2_Simulated79/2
  Merge2_Simulated78/1 -> Merge2_Simulated73/2
  Merge2_Simulated74/1 -> Merge2_Simulated72/2
  Bitmap_Enable11/8 -> Merge2_Simulated121/1
  Bitmap_Enable12/6 -> Merge2_Simulated100/1
  Merge2_Simulated66/1 -> Merge2_Simulated126/2
  Bitmap_Enable14/8 -> Merge2_Simulated123/1
  Bitmap_Enable8/1 -> Merge2_Simulated64/1
  Bitmap_Enable11/5 -> Merge2_Simulated94/1
  Bitmap_Enable10/8 -> Merge2_Simulated119/1
  Bitmap_Enable13/6 -> Merge2_Simulated104/1
  Bitmap_Enable8/5 -> Merge2_Simulated90/1
  Bitmap_Enable14/5 -> Merge2_Simulated96/1
  Bitmap_Enable8/8 -> Merge2_Simulated116/1
  Bitmap_Enable14/2 -> Merge2_Simulated70/1
  Bitmap_Enable12/8 -> Merge2_Simulated117/1
  Bitmap_Enable11/7 -> Merge2_Simulated112/1
  Merge2_Simulated73/1 -> Merge2_Simulated77/2
  Bitmap_Enable10/1 -> Merge2_Simulated87/1
  Bitmap_Enable10/5 -> Merge2_Simulated93/1
  Bitmap_Enable14/3 -> Merge2_Simulated79/1
  Bitmap_Enable13/4 -> Merge2_Simulated86/1
  Bitmap_Enable11/1 -> Merge2_Simulated98/1
  Bitmap_Enable11/6 -> Merge2_Simulated103/1
  Bitmap_Enable10/6 -> Merge2_Simulated102/1
  Merge2_Simulated87/1 -> Merge2_Simulated76/2
  Bitmap_Enable9/4 -> Merge2_Simulated83/1
  Bitmap_Enable9/5 -> Merge2_Simulated92/1
  Bitmap_Enable9/6 -> Merge2_Simulated101/1
  Bitmap_Enable14/4 -> Merge2_Simulated88/1
  Bitmap_Enable14/7 -> Merge2_Simulated114/1
  Bitmap_Enable9/7 -> Merge2_Simulated110/1
  Bitmap_Enable15/1 -> Merge2_Simulated120/2
  Merge2_Simulated120/1 -> Merge2_Simulated109/2
  Bitmap_Enable8/2 -> Merge2_Simulated126/1
  Merge2_Simulated109/1 -> Merge2_Simulated65/2
  Bitmap_Enable9/2 -> Merge2_Simulated66/1
  Bitmap_Enable11/2 -> Merge2_Simulated68/1
  Bitmap_Enable9/8 -> Merge2_Simulated118/1
  Merge2_Simulated67/1 -> Merge2_Simulated66/2
  Merge2_Simulated113/1 -> Merge2_Simulated108/2
  Merge2_Simulated114/1 -> Merge2_Simulated113/2
  Merge2_Simulated108/1 -> Merge2_Simulated112/2
  Merge2_Simulated111/1 -> Merge2_Simulated110/2
  Merge2_Simulated112/1 -> Merge2_Simulated111/2
  Bitmap_Enable8/6 -> Merge2_Simulated99/1
  Bitmap_Enable13/7 -> Merge2_Simulated113/1
  Merge2_Simulated92/1 -> Merge2_Simulated90/2
  Merge2_Simulated95/1 -> Merge2_Simulated91/2
  Merge2_Simulated94/1 -> Merge2_Simulated93/2
  Merge2_Simulated96/1 -> Merge2_Simulated95/2
  Merge2_Simulated76/1 -> Merge2_Simulated64/2
  Merge2_Simulated93/1 -> Merge2_Simulated92/2
  Bitmap_Enable10/3 -> Merge2_Simulated75/1
  Bitmap_Enable14/1 -> Merge2_Simulated120/1
  Bitmap_Enable8/4 -> Merge2_Simulated81/1
  Bitmap_Enable9/3 -> Merge2_Simulated74/1
  Bitmap_Enable12/5 -> Merge2_Simulated91/1
  Merge2_Simulated91/1 -> Merge2_Simulated94/2
  Merge2_Simulated103/1 -> Merge2_Simulated102/2
  Bitmap_Enable15/6 -> Merge2_Simulated105/2
  Bitmap_Enable13/3 -> Merge2_Simulated78/1
  Merge2_Simulated101/1 -> Merge2_Simulated99/2
  Bitmap_Enable13/1 -> Merge2_Simulated109/1
  Bitmap_Enable15/7 -> Merge2_Simulated114/2
  Merge2_Simulated100/1 -> Merge2_Simulated103/2
  Merge2_Simulated105/1 -> Merge2_Simulated104/2
  Merge2_Simulated102/1 -> Merge2_Simulated101/2
  Bitmap_Enable12/1 -> Merge2_Simulated65/1
  Merge2_Simulated117/1 -> Merge2_Simulated121/2
  Bitmap_Enable9/1 -> Merge2_Simulated76/1
  Merge2_Simulated121/1 -> Merge2_Simulated119/2
  Bitmap_Enable10/4 -> Merge2_Simulated84/1
  Bitmap_Enable15/8 -> Merge2_Simulated123/2
  Bitmap_Enable12/4 -> Merge2_Simulated82/1
  Bitmap_Enable8/3 -> Merge2_Simulated72/1
  Merge2_Simulated118/1 -> Merge2_Simulated116/2
  Bitmap_Enable12/7 -> Merge2_Simulated108/1
  Bitmap_Enable13/5 -> Merge2_Simulated95/1
  Merge2_Simulated122/1 -> Merge2_Simulated117/2
  Bitmap_Enable15/5 -> Merge2_Simulated96/2
  Merge2_Simulated65/1 -> Merge2_Simulated98/2
  Merge2_Simulated123/1 -> Merge2_Simulated122/2
  Bitmap_Enable11/4 -> Merge2_Simulated85/1
  Bitmap_Enable12/3 -> Merge2_Simulated73/1
  Bitmap_Enable11/3 -> Merge2_Simulated77/1
  Bitmap_Enable8/7 -> Merge2_Simulated107/1
  Merge2_Simulated85/1 -> Merge2_Simulated84/2
  Merge2_Simulated119/1 -> Merge2_Simulated118/2
  Merge2_Simulated88/1 -> Merge2_Simulated86/2
  Merge2_Simulated98/1 -> Merge2_Simulated87/2
  Merge2_Simulated127/1 -> Merge2_Simulated68/2
  Merge2_Simulated86/1 -> Merge2_Simulated82/2
  Merge2_Simulated83/1 -> Merge2_Simulated81/2
  Merge2_Simulated82/1 -> Merge2_Simulated85/2
  Bitmap_Enable13/8 -> Merge2_Simulated122/1
  Bitmap_Enable12/2 -> Merge2_Simulated127/1
  Merge2_Simulated84/1 -> Merge2_Simulated83/2
  Bitmap_Enable10/7 -> Merge2_Simulated111/1
  Bitmap_Enable13/2 -> Merge2_Simulated69/1
  Merge2_Simulated104/1 -> Merge2_Simulated100/2
  Bitmap_Enable10/2 -> Merge2_Simulated67/1
  Merge2_Simulated110/1 -> Merge2_Simulated107/2
  Bitmap_Enable15/4 -> Merge2_Simulated88/2
  Merge2_Simulated134/1 -> Merge2_Simulated133/2
  Bitmap_Enable23/2 -> Merge2_Simulated134/2
  Merge2_Simulated133/1 -> Merge2_Simulated191/2
  Merge2_Simulated132/1 -> Merge2_Simulated131/2
  Bitmap_Enable22/6 -> Merge2_Simulated169/1
  Merge2_Simulated141/1 -> Merge2_Simulated139/2
  Merge2_Simulated139/1 -> Merge2_Simulated138/2
  Merge2_Simulated143/1 -> Merge2_Simulated142/2
  Bitmap_Enable23/3 -> Merge2_Simulated143/2
  Merge2_Simulated142/1 -> Merge2_Simulated137/2
  Merge2_Simulated138/1 -> Merge2_Simulated136/2
  Bitmap_Enable19/8 -> Merge2_Simulated185/1
  Bitmap_Enable20/6 -> Merge2_Simulated164/1
  Merge2_Simulated130/1 -> Merge2_Simulated190/2
  Bitmap_Enable22/8 -> Merge2_Simulated187/1
  Bitmap_Enable16/1 -> Merge2_Simulated128/1
  Bitmap_Enable19/5 -> Merge2_Simulated158/1
  Bitmap_Enable18/8 -> Merge2_Simulated183/1
  Bitmap_Enable21/6 -> Merge2_Simulated168/1
  Bitmap_Enable16/5 -> Merge2_Simulated154/1
  Bitmap_Enable22/5 -> Merge2_Simulated160/1
  Bitmap_Enable16/8 -> Merge2_Simulated180/1
  Bitmap_Enable22/2 -> Merge2_Simulated134/1
  Bitmap_Enable20/8 -> Merge2_Simulated181/1
  Bitmap_Enable19/7 -> Merge2_Simulated176/1
  Merge2_Simulated137/1 -> Merge2_Simulated141/2
  Bitmap_Enable18/1 -> Merge2_Simulated151/1
  Bitmap_Enable18/5 -> Merge2_Simulated157/1
  Bitmap_Enable22/3 -> Merge2_Simulated143/1
  Bitmap_Enable21/4 -> Merge2_Simulated150/1
  Bitmap_Enable19/1 -> Merge2_Simulated162/1
  Bitmap_Enable19/6 -> Merge2_Simulated167/1
  Bitmap_Enable18/6 -> Merge2_Simulated166/1
  Merge2_Simulated151/1 -> Merge2_Simulated140/2
  Bitmap_Enable17/4 -> Merge2_Simulated147/1
  Bitmap_Enable17/5 -> Merge2_Simulated156/1
  Bitmap_Enable17/6 -> Merge2_Simulated165/1
  Bitmap_Enable22/4 -> Merge2_Simulated152/1
  Bitmap_Enable22/7 -> Merge2_Simulated178/1
  Bitmap_Enable17/7 -> Merge2_Simulated174/1
  Bitmap_Enable23/1 -> Merge2_Simulated184/2
  Merge2_Simulated184/1 -> Merge2_Simulated173/2
  Bitmap_Enable16/2 -> Merge2_Simulated190/1
  Merge2_Simulated173/1 -> Merge2_Simulated129/2
  Bitmap_Enable17/2 -> Merge2_Simulated130/1
  Bitmap_Enable19/2 -> Merge2_Simulated132/1
  Bitmap_Enable17/8 -> Merge2_Simulated182/1
  Merge2_Simulated131/1 -> Merge2_Simulated130/2
  Merge2_Simulated177/1 -> Merge2_Simulated172/2
  Merge2_Simulated178/1 -> Merge2_Simulated177/2
  Merge2_Simulated172/1 -> Merge2_Simulated176/2
  Merge2_Simulated175/1 -> Merge2_Simulated174/2
  Merge2_Simulated176/1 -> Merge2_Simulated175/2
  Bitmap_Enable16/6 -> Merge2_Simulated163/1
  Bitmap_Enable21/7 -> Merge2_Simulated177/1
  Merge2_Simulated156/1 -> Merge2_Simulated154/2
  Merge2_Simulated159/1 -> Merge2_Simulated155/2
  Merge2_Simulated158/1 -> Merge2_Simulated157/2
  Merge2_Simulated160/1 -> Merge2_Simulated159/2
  Merge2_Simulated140/1 -> Merge2_Simulated128/2
  Merge2_Simulated157/1 -> Merge2_Simulated156/2
  Bitmap_Enable18/3 -> Merge2_Simulated139/1
  Bitmap_Enable22/1 -> Merge2_Simulated184/1
  Bitmap_Enable16/4 -> Merge2_Simulated145/1
  Bitmap_Enable17/3 -> Merge2_Simulated138/1
  Bitmap_Enable20/5 -> Merge2_Simulated155/1
  Merge2_Simulated155/1 -> Merge2_Simulated158/2
  Merge2_Simulated167/1 -> Merge2_Simulated166/2
  Bitmap_Enable23/6 -> Merge2_Simulated169/2
  Bitmap_Enable21/3 -> Merge2_Simulated142/1
  Merge2_Simulated165/1 -> Merge2_Simulated163/2
  Bitmap_Enable21/1 -> Merge2_Simulated173/1
  Bitmap_Enable23/7 -> Merge2_Simulated178/2
  Merge2_Simulated164/1 -> Merge2_Simulated167/2
  Merge2_Simulated169/1 -> Merge2_Simulated168/2
  Merge2_Simulated166/1 -> Merge2_Simulated165/2
  Bitmap_Enable20/1 -> Merge2_Simulated129/1
  Merge2_Simulated181/1 -> Merge2_Simulated185/2
  Bitmap_Enable17/1 -> Merge2_Simulated140/1
  Merge2_Simulated185/1 -> Merge2_Simulated183/2
  Bitmap_Enable18/4 -> Merge2_Simulated148/1
  Bitmap_Enable23/8 -> Merge2_Simulated187/2
  Bitmap_Enable20/4 -> Merge2_Simulated146/1
  Bitmap_Enable16/3 -> Merge2_Simulated136/1
  Merge2_Simulated182/1 -> Merge2_Simulated180/2
  Bitmap_Enable20/7 -> Merge2_Simulated172/1
  Bitmap_Enable21/5 -> Merge2_Simulated159/1
  Merge2_Simulated186/1 -> Merge2_Simulated181/2
  Bitmap_Enable23/5 -> Merge2_Simulated160/2
  Merge2_Simulated129/1 -> Merge2_Simulated162/2
  Merge2_Simulated187/1 -> Merge2_Simulated186/2
  Bitmap_Enable19/4 -> Merge2_Simulated149/1
  Bitmap_Enable20/3 -> Merge2_Simulated137/1
  Bitmap_Enable19/3 -> Merge2_Simulated141/1
  Bitmap_Enable16/7 -> Merge2_Simulated171/1
  Merge2_Simulated149/1 -> Merge2_Simulated148/2
  Merge2_Simulated183/1 -> Merge2_Simulated182/2
  Merge2_Simulated152/1 -> Merge2_Simulated150/2
  Merge2_Simulated162/1 -> Merge2_Simulated151/2
  Merge2_Simulated191/1 -> Merge2_Simulated132/2
  Merge2_Simulated150/1 -> Merge2_Simulated146/2
  Merge2_Simulated147/1 -> Merge2_Simulated145/2
  Merge2_Simulated146/1 -> Merge2_Simulated149/2
  Bitmap_Enable21/8 -> Merge2_Simulated186/1
  Bitmap_Enable20/2 -> Merge2_Simulated191/1
  Merge2_Simulated148/1 -> Merge2_Simulated147/2
  Bitmap_Enable18/7 -> Merge2_Simulated175/1
  Bitmap_Enable21/2 -> Merge2_Simulated133/1
  Merge2_Simulated168/1 -> Merge2_Simulated164/2
  Bitmap_Enable18/2 -> Merge2_Simulated131/1
  Merge2_Simulated174/1 -> Merge2_Simulated171/2
  Bitmap_Enable23/4 -> Merge2_Simulated152/2
  Merge2_Simulated198/1 -> Merge2_Simulated197/2
  Bitmap_Enable31/2 -> Merge2_Simulated198/2
  Merge2_Simulated197/1 -> Merge2_Simulated255/2
  Merge2_Simulated196/1 -> Merge2_Simulated195/2
  Bitmap_Enable30/6 -> Merge2_Simulated233/1
  Merge2_Simulated205/1 -> Merge2_Simulated203/2
  Merge2_Simulated203/1 -> Merge2_Simulated202/2
  Merge2_Simulated207/1 -> Merge2_Simulated206/2
  Bitmap_Enable31/3 -> Merge2_Simulated207/2
  Merge2_Simulated206/1 -> Merge2_Simulated201/2
  Merge2_Simulated202/1 -> Merge2_Simulated200/2
  Bitmap_Enable27/8 -> Merge2_Simulated249/1
  Bitmap_Enable28/6 -> Merge2_Simulated228/1
  Merge2_Simulated194/1 -> Merge2_Simulated254/2
  Bitmap_Enable30/8 -> Merge2_Simulated251/1
  Bitmap_Enable24/1 -> Merge2_Simulated192/1
  Bitmap_Enable27/5 -> Merge2_Simulated222/1
  Bitmap_Enable26/8 -> Merge2_Simulated247/1
  Bitmap_Enable29/6 -> Merge2_Simulated232/1
  Bitmap_Enable24/5 -> Merge2_Simulated218/1
  Bitmap_Enable30/5 -> Merge2_Simulated224/1
  Bitmap_Enable24/8 -> Merge2_Simulated244/1
  Bitmap_Enable30/2 -> Merge2_Simulated198/1
  Bitmap_Enable28/8 -> Merge2_Simulated245/1
  Bitmap_Enable27/7 -> Merge2_Simulated240/1
  Merge2_Simulated201/1 -> Merge2_Simulated205/2
  Bitmap_Enable26/1 -> Merge2_Simulated215/1
  Bitmap_Enable26/5 -> Merge2_Simulated221/1
  Bitmap_Enable30/3 -> Merge2_Simulated207/1
  Bitmap_Enable29/4 -> Merge2_Simulated214/1
  Bitmap_Enable27/1 -> Merge2_Simulated226/1
  Bitmap_Enable27/6 -> Merge2_Simulated231/1
  Bitmap_Enable26/6 -> Merge2_Simulated230/1
  Merge2_Simulated215/1 -> Merge2_Simulated204/2
  Bitmap_Enable25/4 -> Merge2_Simulated211/1
  Bitmap_Enable25/5 -> Merge2_Simulated220/1
  Bitmap_Enable25/6 -> Merge2_Simulated229/1
  Bitmap_Enable30/4 -> Merge2_Simulated216/1
  Bitmap_Enable30/7 -> Merge2_Simulated242/1
  Bitmap_Enable25/7 -> Merge2_Simulated238/1
  Bitmap_Enable31/1 -> Merge2_Simulated248/2
  Merge2_Simulated248/1 -> Merge2_Simulated237/2
  Bitmap_Enable24/2 -> Merge2_Simulated254/1
  Merge2_Simulated237/1 -> Merge2_Simulated193/2
  Bitmap_Enable25/2 -> Merge2_Simulated194/1
  Bitmap_Enable27/2 -> Merge2_Simulated196/1
  Bitmap_Enable25/8 -> Merge2_Simulated246/1
  Merge2_Simulated195/1 -> Merge2_Simulated194/2
  Merge2_Simulated241/1 -> Merge2_Simulated236/2
  Merge2_Simulated242/1 -> Merge2_Simulated241/2
  Merge2_Simulated236/1 -> Merge2_Simulated240/2
  Merge2_Simulated239/1 -> Merge2_Simulated238/2
  Merge2_Simulated240/1 -> Merge2_Simulated239/2
  Bitmap_Enable24/6 -> Merge2_Simulated227/1
  Bitmap_Enable29/7 -> Merge2_Simulated241/1
  Merge2_Simulated220/1 -> Merge2_Simulated218/2
  Merge2_Simulated223/1 -> Merge2_Simulated219/2
  Merge2_Simulated222/1 -> Merge2_Simulated221/2
  Merge2_Simulated224/1 -> Merge2_Simulated223/2
  Merge2_Simulated204/1 -> Merge2_Simulated192/2
  Merge2_Simulated221/1 -> Merge2_Simulated220/2
  Bitmap_Enable26/3 -> Merge2_Simulated203/1
  Bitmap_Enable30/1 -> Merge2_Simulated248/1
  Bitmap_Enable24/4 -> Merge2_Simulated209/1
  Bitmap_Enable25/3 -> Merge2_Simulated202/1
  Bitmap_Enable28/5 -> Merge2_Simulated219/1
  Merge2_Simulated219/1 -> Merge2_Simulated222/2
  Merge2_Simulated231/1 -> Merge2_Simulated230/2
  Bitmap_Enable31/6 -> Merge2_Simulated233/2
  Bitmap_Enable29/3 -> Merge2_Simulated206/1
  Merge2_Simulated229/1 -> Merge2_Simulated227/2
  Bitmap_Enable29/1 -> Merge2_Simulated237/1
  Bitmap_Enable31/7 -> Merge2_Simulated242/2
  Merge2_Simulated228/1 -> Merge2_Simulated231/2
  Merge2_Simulated233/1 -> Merge2_Simulated232/2
  Merge2_Simulated230/1 -> Merge2_Simulated229/2
  Bitmap_Enable28/1 -> Merge2_Simulated193/1
  Merge2_Simulated245/1 -> Merge2_Simulated249/2
  Bitmap_Enable25/1 -> Merge2_Simulated204/1
  Merge2_Simulated249/1 -> Merge2_Simulated247/2
  Bitmap_Enable26/4 -> Merge2_Simulated212/1
  Bitmap_Enable31/8 -> Merge2_Simulated251/2
  Bitmap_Enable28/4 -> Merge2_Simulated210/1
  Bitmap_Enable24/3 -> Merge2_Simulated200/1
  Merge2_Simulated246/1 -> Merge2_Simulated244/2
  Bitmap_Enable28/7 -> Merge2_Simulated236/1
  Bitmap_Enable29/5 -> Merge2_Simulated223/1
  Merge2_Simulated250/1 -> Merge2_Simulated245/2
  Bitmap_Enable31/5 -> Merge2_Simulated224/2
  Merge2_Simulated193/1 -> Merge2_Simulated226/2
  Merge2_Simulated251/1 -> Merge2_Simulated250/2
  Bitmap_Enable27/4 -> Merge2_Simulated213/1
  Bitmap_Enable28/3 -> Merge2_Simulated201/1
  Bitmap_Enable27/3 -> Merge2_Simulated205/1
  Bitmap_Enable24/7 -> Merge2_Simulated235/1
  Merge2_Simulated213/1 -> Merge2_Simulated212/2
  Merge2_Simulated247/1 -> Merge2_Simulated246/2
  Merge2_Simulated216/1 -> Merge2_Simulated214/2
  Merge2_Simulated226/1 -> Merge2_Simulated215/2
  Merge2_Simulated255/1 -> Merge2_Simulated196/2
  Merge2_Simulated214/1 -> Merge2_Simulated210/2
  Merge2_Simulated211/1 -> Merge2_Simulated209/2
  Merge2_Simulated210/1 -> Merge2_Simulated213/2
  Bitmap_Enable29/8 -> Merge2_Simulated250/1
  Bitmap_Enable28/2 -> Merge2_Simulated255/1
  Merge2_Simulated212/1 -> Merge2_Simulated211/2
  Bitmap_Enable26/7 -> Merge2_Simulated239/1
  Bitmap_Enable29/2 -> Merge2_Simulated197/1
  Merge2_Simulated232/1 -> Merge2_Simulated228/2
  Bitmap_Enable26/2 -> Merge2_Simulated195/1
  Merge2_Simulated238/1 -> Merge2_Simulated235/2
  Bitmap_Enable31/4 -> Merge2_Simulated216/2
  Merge2_Simulated262/1 -> Merge2_Simulated261/2
  Bitmap_Enable39/2 -> Merge2_Simulated262/2
  Merge2_Simulated261/1 -> Merge2_Simulated319/2
  Merge2_Simulated260/1 -> Merge2_Simulated259/2
  Bitmap_Enable38/6 -> Merge2_Simulated297/1
  Merge2_Simulated269/1 -> Merge2_Simulated267/2
  Merge2_Simulated267/1 -> Merge2_Simulated266/2
  Merge2_Simulated271/1 -> Merge2_Simulated270/2
  Bitmap_Enable39/3 -> Merge2_Simulated271/2
  Merge2_Simulated270/1 -> Merge2_Simulated265/2
  Merge2_Simulated266/1 -> Merge2_Simulated264/2
  Bitmap_Enable35/8 -> Merge2_Simulated313/1
  Bitmap_Enable36/6 -> Merge2_Simulated292/1
  Merge2_Simulated258/1 -> Merge2_Simulated318/2
  Bitmap_Enable38/8 -> Merge2_Simulated315/1
  Bitmap_Enable32/1 -> Merge2_Simulated256/1
  Bitmap_Enable35/5 -> Merge2_Simulated286/1
  Bitmap_Enable34/8 -> Merge2_Simulated311/1
  Bitmap_Enable37/6 -> Merge2_Simulated296/1
  Bitmap_Enable32/5 -> Merge2_Simulated282/1
  Bitmap_Enable38/5 -> Merge2_Simulated288/1
  Bitmap_Enable32/8 -> Merge2_Simulated308/1
  Bitmap_Enable38/2 -> Merge2_Simulated262/1
  Bitmap_Enable36/8 -> Merge2_Simulated309/1
  Bitmap_Enable35/7 -> Merge2_Simulated304/1
  Merge2_Simulated265/1 -> Merge2_Simulated269/2
  Bitmap_Enable34/1 -> Merge2_Simulated279/1
  Bitmap_Enable34/5 -> Merge2_Simulated285/1
  Bitmap_Enable38/3 -> Merge2_Simulated271/1
  Bitmap_Enable37/4 -> Merge2_Simulated278/1
  Bitmap_Enable35/1 -> Merge2_Simulated290/1
  Bitmap_Enable35/6 -> Merge2_Simulated295/1
  Bitmap_Enable34/6 -> Merge2_Simulated294/1
  Merge2_Simulated279/1 -> Merge2_Simulated268/2
  Bitmap_Enable33/4 -> Merge2_Simulated275/1
  Bitmap_Enable33/5 -> Merge2_Simulated284/1
  Bitmap_Enable33/6 -> Merge2_Simulated293/1
  Bitmap_Enable38/4 -> Merge2_Simulated280/1
  Bitmap_Enable38/7 -> Merge2_Simulated306/1
  Bitmap_Enable33/7 -> Merge2_Simulated302/1
  Bitmap_Enable39/1 -> Merge2_Simulated312/2
  Merge2_Simulated312/1 -> Merge2_Simulated301/2
  Bitmap_Enable32/2 -> Merge2_Simulated318/1
  Merge2_Simulated301/1 -> Merge2_Simulated257/2
  Bitmap_Enable33/2 -> Merge2_Simulated258/1
  Bitmap_Enable35/2 -> Merge2_Simulated260/1
  Bitmap_Enable33/8 -> Merge2_Simulated310/1
  Merge2_Simulated259/1 -> Merge2_Simulated258/2
  Merge2_Simulated305/1 -> Merge2_Simulated300/2
  Merge2_Simulated306/1 -> Merge2_Simulated305/2
  Merge2_Simulated300/1 -> Merge2_Simulated304/2
  Merge2_Simulated303/1 -> Merge2_Simulated302/2
  Merge2_Simulated304/1 -> Merge2_Simulated303/2
  Bitmap_Enable32/6 -> Merge2_Simulated291/1
  Bitmap_Enable37/7 -> Merge2_Simulated305/1
  Merge2_Simulated284/1 -> Merge2_Simulated282/2
  Merge2_Simulated287/1 -> Merge2_Simulated283/2
  Merge2_Simulated286/1 -> Merge2_Simulated285/2
  Merge2_Simulated288/1 -> Merge2_Simulated287/2
  Merge2_Simulated268/1 -> Merge2_Simulated256/2
  Merge2_Simulated285/1 -> Merge2_Simulated284/2
  Bitmap_Enable34/3 -> Merge2_Simulated267/1
  Bitmap_Enable38/1 -> Merge2_Simulated312/1
  Bitmap_Enable32/4 -> Merge2_Simulated273/1
  Bitmap_Enable33/3 -> Merge2_Simulated266/1
  Bitmap_Enable36/5 -> Merge2_Simulated283/1
  Merge2_Simulated283/1 -> Merge2_Simulated286/2
  Merge2_Simulated295/1 -> Merge2_Simulated294/2
  Bitmap_Enable39/6 -> Merge2_Simulated297/2
  Bitmap_Enable37/3 -> Merge2_Simulated270/1
  Merge2_Simulated293/1 -> Merge2_Simulated291/2
  Bitmap_Enable37/1 -> Merge2_Simulated301/1
  Bitmap_Enable39/7 -> Merge2_Simulated306/2
  Merge2_Simulated292/1 -> Merge2_Simulated295/2
  Merge2_Simulated297/1 -> Merge2_Simulated296/2
  Merge2_Simulated294/1 -> Merge2_Simulated293/2
  Bitmap_Enable36/1 -> Merge2_Simulated257/1
  Merge2_Simulated309/1 -> Merge2_Simulated313/2
  Bitmap_Enable33/1 -> Merge2_Simulated268/1
  Merge2_Simulated313/1 -> Merge2_Simulated311/2
  Bitmap_Enable34/4 -> Merge2_Simulated276/1
  Bitmap_Enable39/8 -> Merge2_Simulated315/2
  Bitmap_Enable36/4 -> Merge2_Simulated274/1
  Bitmap_Enable32/3 -> Merge2_Simulated264/1
  Merge2_Simulated310/1 -> Merge2_Simulated308/2
  Bitmap_Enable36/7 -> Merge2_Simulated300/1
  Bitmap_Enable37/5 -> Merge2_Simulated287/1
  Merge2_Simulated314/1 -> Merge2_Simulated309/2
  Bitmap_Enable39/5 -> Merge2_Simulated288/2
  Merge2_Simulated257/1 -> Merge2_Simulated290/2
  Merge2_Simulated315/1 -> Merge2_Simulated314/2
  Bitmap_Enable35/4 -> Merge2_Simulated277/1
  Bitmap_Enable36/3 -> Merge2_Simulated265/1
  Bitmap_Enable35/3 -> Merge2_Simulated269/1
  Bitmap_Enable32/7 -> Merge2_Simulated299/1
  Merge2_Simulated277/1 -> Merge2_Simulated276/2
  Merge2_Simulated311/1 -> Merge2_Simulated310/2
  Merge2_Simulated280/1 -> Merge2_Simulated278/2
  Merge2_Simulated290/1 -> Merge2_Simulated279/2
  Merge2_Simulated319/1 -> Merge2_Simulated260/2
  Merge2_Simulated278/1 -> Merge2_Simulated274/2
  Merge2_Simulated275/1 -> Merge2_Simulated273/2
  Merge2_Simulated274/1 -> Merge2_Simulated277/2
  Bitmap_Enable37/8 -> Merge2_Simulated314/1
  Bitmap_Enable36/2 -> Merge2_Simulated319/1
  Merge2_Simulated276/1 -> Merge2_Simulated275/2
  Bitmap_Enable34/7 -> Merge2_Simulated303/1
  Bitmap_Enable37/2 -> Merge2_Simulated261/1
  Merge2_Simulated296/1 -> Merge2_Simulated292/2
  Bitmap_Enable34/2 -> Merge2_Simulated259/1
  Merge2_Simulated302/1 -> Merge2_Simulated299/2
  Bitmap_Enable39/4 -> Merge2_Simulated280/2
  Merge2_Simulated326/1 -> Merge2_Simulated325/2
  Bitmap_Enable47/2 -> Merge2_Simulated326/2
  Merge2_Simulated325/1 -> Merge2_Simulated383/2
  Merge2_Simulated324/1 -> Merge2_Simulated323/2
  Bitmap_Enable46/6 -> Merge2_Simulated361/1
  Merge2_Simulated333/1 -> Merge2_Simulated331/2
  Merge2_Simulated331/1 -> Merge2_Simulated330/2
  Merge2_Simulated335/1 -> Merge2_Simulated334/2
  Bitmap_Enable47/3 -> Merge2_Simulated335/2
  Merge2_Simulated334/1 -> Merge2_Simulated329/2
  Merge2_Simulated330/1 -> Merge2_Simulated328/2
  Bitmap_Enable43/8 -> Merge2_Simulated377/1
  Bitmap_Enable44/6 -> Merge2_Simulated356/1
  Merge2_Simulated322/1 -> Merge2_Simulated382/2
  Bitmap_Enable46/8 -> Merge2_Simulated379/1
  Bitmap_Enable40/1 -> Merge2_Simulated320/1
  Bitmap_Enable43/5 -> Merge2_Simulated350/1
  Bitmap_Enable42/8 -> Merge2_Simulated375/1
  Bitmap_Enable45/6 -> Merge2_Simulated360/1
  Bitmap_Enable40/5 -> Merge2_Simulated346/1
  Bitmap_Enable46/5 -> Merge2_Simulated352/1
  Bitmap_Enable40/8 -> Merge2_Simulated372/1
  Bitmap_Enable46/2 -> Merge2_Simulated326/1
  Bitmap_Enable44/8 -> Merge2_Simulated373/1
  Bitmap_Enable43/7 -> Merge2_Simulated368/1
  Merge2_Simulated329/1 -> Merge2_Simulated333/2
  Bitmap_Enable42/1 -> Merge2_Simulated343/1
  Bitmap_Enable42/5 -> Merge2_Simulated349/1
  Bitmap_Enable46/3 -> Merge2_Simulated335/1
  Bitmap_Enable45/4 -> Merge2_Simulated342/1
  Bitmap_Enable43/1 -> Merge2_Simulated354/1
  Bitmap_Enable43/6 -> Merge2_Simulated359/1
  Bitmap_Enable42/6 -> Merge2_Simulated358/1
  Merge2_Simulated343/1 -> Merge2_Simulated332/2
  Bitmap_Enable41/4 -> Merge2_Simulated339/1
  Bitmap_Enable41/5 -> Merge2_Simulated348/1
  Bitmap_Enable41/6 -> Merge2_Simulated357/1
  Bitmap_Enable46/4 -> Merge2_Simulated344/1
  Bitmap_Enable46/7 -> Merge2_Simulated370/1
  Bitmap_Enable41/7 -> Merge2_Simulated366/1
  Bitmap_Enable47/1 -> Merge2_Simulated376/2
  Merge2_Simulated376/1 -> Merge2_Simulated365/2
  Bitmap_Enable40/2 -> Merge2_Simulated382/1
  Merge2_Simulated365/1 -> Merge2_Simulated321/2
  Bitmap_Enable41/2 -> Merge2_Simulated322/1
  Bitmap_Enable43/2 -> Merge2_Simulated324/1
  Bitmap_Enable41/8 -> Merge2_Simulated374/1
  Merge2_Simulated323/1 -> Merge2_Simulated322/2
  Merge2_Simulated369/1 -> Merge2_Simulated364/2
  Merge2_Simulated370/1 -> Merge2_Simulated369/2
  Merge2_Simulated364/1 -> Merge2_Simulated368/2
  Merge2_Simulated367/1 -> Merge2_Simulated366/2
  Merge2_Simulated368/1 -> Merge2_Simulated367/2
  Bitmap_Enable40/6 -> Merge2_Simulated355/1
  Bitmap_Enable45/7 -> Merge2_Simulated369/1
  Merge2_Simulated348/1 -> Merge2_Simulated346/2
  Merge2_Simulated351/1 -> Merge2_Simulated347/2
  Merge2_Simulated350/1 -> Merge2_Simulated349/2
  Merge2_Simulated352/1 -> Merge2_Simulated351/2
  Merge2_Simulated332/1 -> Merge2_Simulated320/2
  Merge2_Simulated349/1 -> Merge2_Simulated348/2
  Bitmap_Enable42/3 -> Merge2_Simulated331/1
  Bitmap_Enable46/1 -> Merge2_Simulated376/1
  Bitmap_Enable40/4 -> Merge2_Simulated337/1
  Bitmap_Enable41/3 -> Merge2_Simulated330/1
  Bitmap_Enable44/5 -> Merge2_Simulated347/1
  Merge2_Simulated347/1 -> Merge2_Simulated350/2
  Merge2_Simulated359/1 -> Merge2_Simulated358/2
  Bitmap_Enable47/6 -> Merge2_Simulated361/2
  Bitmap_Enable45/3 -> Merge2_Simulated334/1
  Merge2_Simulated357/1 -> Merge2_Simulated355/2
  Bitmap_Enable45/1 -> Merge2_Simulated365/1
  Bitmap_Enable47/7 -> Merge2_Simulated370/2
  Merge2_Simulated356/1 -> Merge2_Simulated359/2
  Merge2_Simulated361/1 -> Merge2_Simulated360/2
  Merge2_Simulated358/1 -> Merge2_Simulated357/2
  Bitmap_Enable44/1 -> Merge2_Simulated321/1
  Merge2_Simulated373/1 -> Merge2_Simulated377/2
  Bitmap_Enable41/1 -> Merge2_Simulated332/1
  Merge2_Simulated377/1 -> Merge2_Simulated375/2
  Bitmap_Enable42/4 -> Merge2_Simulated340/1
  Bitmap_Enable47/8 -> Merge2_Simulated379/2
  Bitmap_Enable44/4 -> Merge2_Simulated338/1
  Bitmap_Enable40/3 -> Merge2_Simulated328/1
  Merge2_Simulated374/1 -> Merge2_Simulated372/2
  Bitmap_Enable44/7 -> Merge2_Simulated364/1
  Bitmap_Enable45/5 -> Merge2_Simulated351/1
  Merge2_Simulated378/1 -> Merge2_Simulated373/2
  Bitmap_Enable47/5 -> Merge2_Simulated352/2
  Merge2_Simulated321/1 -> Merge2_Simulated354/2
  Merge2_Simulated379/1 -> Merge2_Simulated378/2
  Bitmap_Enable43/4 -> Merge2_Simulated341/1
  Bitmap_Enable44/3 -> Merge2_Simulated329/1
  Bitmap_Enable43/3 -> Merge2_Simulated333/1
  Bitmap_Enable40/7 -> Merge2_Simulated363/1
  Merge2_Simulated341/1 -> Merge2_Simulated340/2
  Merge2_Simulated375/1 -> Merge2_Simulated374/2
  Merge2_Simulated344/1 -> Merge2_Simulated342/2
  Merge2_Simulated354/1 -> Merge2_Simulated343/2
  Merge2_Simulated383/1 -> Merge2_Simulated324/2
  Merge2_Simulated342/1 -> Merge2_Simulated338/2
  Merge2_Simulated339/1 -> Merge2_Simulated337/2
  Merge2_Simulated338/1 -> Merge2_Simulated341/2
  Bitmap_Enable45/8 -> Merge2_Simulated378/1
  Bitmap_Enable44/2 -> Merge2_Simulated383/1
  Merge2_Simulated340/1 -> Merge2_Simulated339/2
  Bitmap_Enable42/7 -> Merge2_Simulated367/1
  Bitmap_Enable45/2 -> Merge2_Simulated325/1
  Merge2_Simulated360/1 -> Merge2_Simulated356/2
  Bitmap_Enable42/2 -> Merge2_Simulated323/1
  Merge2_Simulated366/1 -> Merge2_Simulated363/2
  Bitmap_Enable47/4 -> Merge2_Simulated344/2
  Merge2_Simulated390/1 -> Merge2_Simulated389/2
  Bitmap_Enable55/2 -> Merge2_Simulated390/2
  Merge2_Simulated389/1 -> Merge2_Simulated447/2
  Merge2_Simulated388/1 -> Merge2_Simulated387/2
  Bitmap_Enable54/6 -> Merge2_Simulated425/1
  Merge2_Simulated397/1 -> Merge2_Simulated395/2
  Merge2_Simulated395/1 -> Merge2_Simulated394/2
  Merge2_Simulated399/1 -> Merge2_Simulated398/2
  Bitmap_Enable55/3 -> Merge2_Simulated399/2
  Merge2_Simulated398/1 -> Merge2_Simulated393/2
  Merge2_Simulated394/1 -> Merge2_Simulated392/2
  Bitmap_Enable51/8 -> Merge2_Simulated441/1
  Bitmap_Enable52/6 -> Merge2_Simulated420/1
  Merge2_Simulated386/1 -> Merge2_Simulated446/2
  Bitmap_Enable54/8 -> Merge2_Simulated443/1
  Bitmap_Enable48/1 -> Merge2_Simulated384/1
  Bitmap_Enable51/5 -> Merge2_Simulated414/1
  Bitmap_Enable50/8 -> Merge2_Simulated439/1
  Bitmap_Enable53/6 -> Merge2_Simulated424/1
  Bitmap_Enable48/5 -> Merge2_Simulated410/1
  Bitmap_Enable54/5 -> Merge2_Simulated416/1
  Bitmap_Enable48/8 -> Merge2_Simulated436/1
  Bitmap_Enable54/2 -> Merge2_Simulated390/1
  Bitmap_Enable52/8 -> Merge2_Simulated437/1
  Bitmap_Enable51/7 -> Merge2_Simulated432/1
  Merge2_Simulated393/1 -> Merge2_Simulated397/2
  Bitmap_Enable50/1 -> Merge2_Simulated407/1
  Bitmap_Enable50/5 -> Merge2_Simulated413/1
  Bitmap_Enable54/3 -> Merge2_Simulated399/1
  Bitmap_Enable53/4 -> Merge2_Simulated406/1
  Bitmap_Enable51/1 -> Merge2_Simulated418/1
  Bitmap_Enable51/6 -> Merge2_Simulated423/1
  Bitmap_Enable50/6 -> Merge2_Simulated422/1
  Merge2_Simulated407/1 -> Merge2_Simulated396/2
  Bitmap_Enable49/4 -> Merge2_Simulated403/1
  Bitmap_Enable49/5 -> Merge2_Simulated412/1
  Bitmap_Enable49/6 -> Merge2_Simulated421/1
  Bitmap_Enable54/4 -> Merge2_Simulated408/1
  Bitmap_Enable54/7 -> Merge2_Simulated434/1
  Bitmap_Enable49/7 -> Merge2_Simulated430/1
  Bitmap_Enable55/1 -> Merge2_Simulated440/2
  Merge2_Simulated440/1 -> Merge2_Simulated429/2
  Bitmap_Enable48/2 -> Merge2_Simulated446/1
  Merge2_Simulated429/1 -> Merge2_Simulated385/2
  Bitmap_Enable49/2 -> Merge2_Simulated386/1
  Bitmap_Enable51/2 -> Merge2_Simulated388/1
  Bitmap_Enable49/8 -> Merge2_Simulated438/1
  Merge2_Simulated387/1 -> Merge2_Simulated386/2
  Merge2_Simulated433/1 -> Merge2_Simulated428/2
  Merge2_Simulated434/1 -> Merge2_Simulated433/2
  Merge2_Simulated428/1 -> Merge2_Simulated432/2
  Merge2_Simulated431/1 -> Merge2_Simulated430/2
  Merge2_Simulated432/1 -> Merge2_Simulated431/2
  Bitmap_Enable48/6 -> Merge2_Simulated419/1
  Bitmap_Enable53/7 -> Merge2_Simulated433/1
  Merge2_Simulated412/1 -> Merge2_Simulated410/2
  Merge2_Simulated415/1 -> Merge2_Simulated411/2
  Merge2_Simulated414/1 -> Merge2_Simulated413/2
  Merge2_Simulated416/1 -> Merge2_Simulated415/2
  Merge2_Simulated396/1 -> Merge2_Simulated384/2
  Merge2_Simulated413/1 -> Merge2_Simulated412/2
  Bitmap_Enable50/3 -> Merge2_Simulated395/1
  Bitmap_Enable54/1 -> Merge2_Simulated440/1
  Bitmap_Enable48/4 -> Merge2_Simulated401/1
  Bitmap_Enable49/3 -> Merge2_Simulated394/1
  Bitmap_Enable52/5 -> Merge2_Simulated411/1
  Merge2_Simulated411/1 -> Merge2_Simulated414/2
  Merge2_Simulated423/1 -> Merge2_Simulated422/2
  Bitmap_Enable55/6 -> Merge2_Simulated425/2
  Bitmap_Enable53/3 -> Merge2_Simulated398/1
  Merge2_Simulated421/1 -> Merge2_Simulated419/2
  Bitmap_Enable53/1 -> Merge2_Simulated429/1
  Bitmap_Enable55/7 -> Merge2_Simulated434/2
  Merge2_Simulated420/1 -> Merge2_Simulated423/2
  Merge2_Simulated425/1 -> Merge2_Simulated424/2
  Merge2_Simulated422/1 -> Merge2_Simulated421/2
  Bitmap_Enable52/1 -> Merge2_Simulated385/1
  Merge2_Simulated437/1 -> Merge2_Simulated441/2
  Bitmap_Enable49/1 -> Merge2_Simulated396/1
  Merge2_Simulated441/1 -> Merge2_Simulated439/2
  Bitmap_Enable50/4 -> Merge2_Simulated404/1
  Bitmap_Enable55/8 -> Merge2_Simulated443/2
  Bitmap_Enable52/4 -> Merge2_Simulated402/1
  Bitmap_Enable48/3 -> Merge2_Simulated392/1
  Merge2_Simulated438/1 -> Merge2_Simulated436/2
  Bitmap_Enable52/7 -> Merge2_Simulated428/1
  Bitmap_Enable53/5 -> Merge2_Simulated415/1
  Merge2_Simulated442/1 -> Merge2_Simulated437/2
  Bitmap_Enable55/5 -> Merge2_Simulated416/2
  Merge2_Simulated385/1 -> Merge2_Simulated418/2
  Merge2_Simulated443/1 -> Merge2_Simulated442/2
  Bitmap_Enable51/4 -> Merge2_Simulated405/1
  Bitmap_Enable52/3 -> Merge2_Simulated393/1
  Bitmap_Enable51/3 -> Merge2_Simulated397/1
  Bitmap_Enable48/7 -> Merge2_Simulated427/1
  Merge2_Simulated405/1 -> Merge2_Simulated404/2
  Merge2_Simulated439/1 -> Merge2_Simulated438/2
  Merge2_Simulated408/1 -> Merge2_Simulated406/2
  Merge2_Simulated418/1 -> Merge2_Simulated407/2
  Merge2_Simulated447/1 -> Merge2_Simulated388/2
  Merge2_Simulated406/1 -> Merge2_Simulated402/2
  Merge2_Simulated403/1 -> Merge2_Simulated401/2
  Merge2_Simulated402/1 -> Merge2_Simulated405/2
  Bitmap_Enable53/8 -> Merge2_Simulated442/1
  Bitmap_Enable52/2 -> Merge2_Simulated447/1
  Merge2_Simulated404/1 -> Merge2_Simulated403/2
  Bitmap_Enable50/7 -> Merge2_Simulated431/1
  Bitmap_Enable53/2 -> Merge2_Simulated389/1
  Merge2_Simulated424/1 -> Merge2_Simulated420/2
  Bitmap_Enable50/2 -> Merge2_Simulated387/1
  Merge2_Simulated430/1 -> Merge2_Simulated427/2
  Bitmap_Enable55/4 -> Merge2_Simulated408/2
  Merge2_Simulated454/1 -> Merge2_Simulated453/2
  Bitmap_Enable63/2 -> Merge2_Simulated454/2
  Merge2_Simulated453/1 -> Merge2_Simulated511/2
  Merge2_Simulated452/1 -> Merge2_Simulated451/2
  Bitmap_Enable62/6 -> Merge2_Simulated489/1
  Merge2_Simulated461/1 -> Merge2_Simulated459/2
  Merge2_Simulated459/1 -> Merge2_Simulated458/2
  Merge2_Simulated463/1 -> Merge2_Simulated462/2
  Bitmap_Enable63/3 -> Merge2_Simulated463/2
  Merge2_Simulated462/1 -> Merge2_Simulated457/2
  Merge2_Simulated458/1 -> Merge2_Simulated456/2
  Bitmap_Enable59/8 -> Merge2_Simulated505/1
  Bitmap_Enable60/6 -> Merge2_Simulated484/1
  Merge2_Simulated450/1 -> Merge2_Simulated510/2
  Bitmap_Enable62/8 -> Merge2_Simulated507/1
  Bitmap_Enable56/1 -> Merge2_Simulated448/1
  Bitmap_Enable59/5 -> Merge2_Simulated478/1
  Bitmap_Enable58/8 -> Merge2_Simulated503/1
  Bitmap_Enable61/6 -> Merge2_Simulated488/1
  Bitmap_Enable56/5 -> Merge2_Simulated474/1
  Bitmap_Enable62/5 -> Merge2_Simulated480/1
  Bitmap_Enable56/8 -> Merge2_Simulated500/1
  Bitmap_Enable62/2 -> Merge2_Simulated454/1
  Bitmap_Enable60/8 -> Merge2_Simulated501/1
  Bitmap_Enable59/7 -> Merge2_Simulated496/1
  Merge2_Simulated457/1 -> Merge2_Simulated461/2
  Bitmap_Enable58/1 -> Merge2_Simulated471/1
  Bitmap_Enable58/5 -> Merge2_Simulated477/1
  Bitmap_Enable62/3 -> Merge2_Simulated463/1
  Bitmap_Enable61/4 -> Merge2_Simulated470/1
  Bitmap_Enable59/1 -> Merge2_Simulated482/1
  Bitmap_Enable59/6 -> Merge2_Simulated487/1
  Bitmap_Enable58/6 -> Merge2_Simulated486/1
  Merge2_Simulated471/1 -> Merge2_Simulated460/2
  Bitmap_Enable57/4 -> Merge2_Simulated467/1
  Bitmap_Enable57/5 -> Merge2_Simulated476/1
  Bitmap_Enable57/6 -> Merge2_Simulated485/1
  Bitmap_Enable62/4 -> Merge2_Simulated472/1
  Bitmap_Enable62/7 -> Merge2_Simulated498/1
  Bitmap_Enable57/7 -> Merge2_Simulated494/1
  Bitmap_Enable63/1 -> Merge2_Simulated504/2
  Merge2_Simulated504/1 -> Merge2_Simulated493/2
  Bitmap_Enable56/2 -> Merge2_Simulated510/1
  Merge2_Simulated493/1 -> Merge2_Simulated449/2
  Bitmap_Enable57/2 -> Merge2_Simulated450/1
  Bitmap_Enable59/2 -> Merge2_Simulated452/1
  Bitmap_Enable57/8 -> Merge2_Simulated502/1
  Merge2_Simulated451/1 -> Merge2_Simulated450/2
  Merge2_Simulated497/1 -> Merge2_Simulated492/2
  Merge2_Simulated498/1 -> Merge2_Simulated497/2
  Merge2_Simulated492/1 -> Merge2_Simulated496/2
  Merge2_Simulated495/1 -> Merge2_Simulated494/2
  Merge2_Simulated496/1 -> Merge2_Simulated495/2
  Bitmap_Enable56/6 -> Merge2_Simulated483/1
  Bitmap_Enable61/7 -> Merge2_Simulated497/1
  Merge2_Simulated476/1 -> Merge2_Simulated474/2
  Merge2_Simulated479/1 -> Merge2_Simulated475/2
  Merge2_Simulated478/1 -> Merge2_Simulated477/2
  Merge2_Simulated480/1 -> Merge2_Simulated479/2
  Merge2_Simulated460/1 -> Merge2_Simulated448/2
  Merge2_Simulated477/1 -> Merge2_Simulated476/2
  Bitmap_Enable58/3 -> Merge2_Simulated459/1
  Bitmap_Enable62/1 -> Merge2_Simulated504/1
  Bitmap_Enable56/4 -> Merge2_Simulated465/1
  Bitmap_Enable57/3 -> Merge2_Simulated458/1
  Bitmap_Enable60/5 -> Merge2_Simulated475/1
  Merge2_Simulated475/1 -> Merge2_Simulated478/2
  Merge2_Simulated487/1 -> Merge2_Simulated486/2
  Bitmap_Enable63/6 -> Merge2_Simulated489/2
  Bitmap_Enable61/3 -> Merge2_Simulated462/1
  Merge2_Simulated485/1 -> Merge2_Simulated483/2
  Bitmap_Enable61/1 -> Merge2_Simulated493/1
  Bitmap_Enable63/7 -> Merge2_Simulated498/2
  Merge2_Simulated484/1 -> Merge2_Simulated487/2
  Merge2_Simulated489/1 -> Merge2_Simulated488/2
  Merge2_Simulated486/1 -> Merge2_Simulated485/2
  Bitmap_Enable60/1 -> Merge2_Simulated449/1
  Merge2_Simulated501/1 -> Merge2_Simulated505/2
  Bitmap_Enable57/1 -> Merge2_Simulated460/1
  Merge2_Simulated505/1 -> Merge2_Simulated503/2
  Bitmap_Enable58/4 -> Merge2_Simulated468/1
  Bitmap_Enable63/8 -> Merge2_Simulated507/2
  Bitmap_Enable60/4 -> Merge2_Simulated466/1
  Bitmap_Enable56/3 -> Merge2_Simulated456/1
  Merge2_Simulated502/1 -> Merge2_Simulated500/2
  Bitmap_Enable60/7 -> Merge2_Simulated492/1
  Bitmap_Enable61/5 -> Merge2_Simulated479/1
  Merge2_Simulated506/1 -> Merge2_Simulated501/2
  Bitmap_Enable63/5 -> Merge2_Simulated480/2
  Merge2_Simulated449/1 -> Merge2_Simulated482/2
  Merge2_Simulated507/1 -> Merge2_Simulated506/2
  Bitmap_Enable59/4 -> Merge2_Simulated469/1
  Bitmap_Enable60/3 -> Merge2_Simulated457/1
  Bitmap_Enable59/3 -> Merge2_Simulated461/1
  Bitmap_Enable56/7 -> Merge2_Simulated491/1
  Merge2_Simulated469/1 -> Merge2_Simulated468/2
  Merge2_Simulated503/1 -> Merge2_Simulated502/2
  Merge2_Simulated472/1 -> Merge2_Simulated470/2
  Merge2_Simulated482/1 -> Merge2_Simulated471/2
  Merge2_Simulated511/1 -> Merge2_Simulated452/2
  Merge2_Simulated470/1 -> Merge2_Simulated466/2
  Merge2_Simulated467/1 -> Merge2_Simulated465/2
  Merge2_Simulated466/1 -> Merge2_Simulated469/2
  Bitmap_Enable61/8 -> Merge2_Simulated506/1
  Bitmap_Enable60/2 -> Merge2_Simulated511/1
  Merge2_Simulated468/1 -> Merge2_Simulated467/2
  Bitmap_Enable58/7 -> Merge2_Simulated495/1
  Bitmap_Enable61/2 -> Merge2_Simulated453/1
  Merge2_Simulated488/1 -> Merge2_Simulated484/2
  Bitmap_Enable58/2 -> Merge2_Simulated451/1
  Merge2_Simulated494/1 -> Merge2_Simulated491/2
  Bitmap_Enable63/4 -> Merge2_Simulated472/2
  Merge2_Simulated56/1 -> Merge2_Simulated518/2
  Merge2_Simulated116/1 -> Merge2_Simulated518/1
  Merge2_Simulated/1 -> Merge2_Simulated519/2
  Merge2_Simulated8/1 -> Merge2_Simulated517/2
  Merge2_Simulated16/1 -> Merge2_Simulated516/2
  Merge2_Simulated24/1 -> Merge2_Simulated515/2
  Merge2_Simulated32/1 -> Merge2_Simulated514/2
  Merge2_Simulated40/1 -> Merge2_Simulated513/2
  Merge2_Simulated48/1 -> Merge2_Simulated512/2
  Merge2_Simulated64/1 -> Merge2_Simulated519/1
  Merge2_Simulated126/1 -> Merge2_Simulated517/1
  Merge2_Simulated72/1 -> Merge2_Simulated516/1
  Merge2_Simulated81/1 -> Merge2_Simulated515/1
  Merge2_Simulated90/1 -> Merge2_Simulated514/1
  Merge2_Simulated99/1 -> Merge2_Simulated513/1
  Merge2_Simulated107/1 -> Merge2_Simulated512/1
  Merge2_Simulated128/1 -> Merge2_Simulated527/1
  Merge2_Simulated163/1 -> Merge2_Simulated521/1
  Merge2_Simulated145/1 -> Merge2_Simulated523/1
  Merge2_Simulated190/1 -> Merge2_Simulated525/1
  Merge2_Simulated154/1 -> Merge2_Simulated522/1
  Merge2_Simulated180/1 -> Merge2_Simulated526/1
  Merge2_Simulated171/1 -> Merge2_Simulated520/1
  Merge2_Simulated136/1 -> Merge2_Simulated524/1
  Merge2_Simulated519/1 -> Merge2_Simulated527/2
  Merge2_Simulated517/1 -> Merge2_Simulated525/2
  Merge2_Simulated516/1 -> Merge2_Simulated524/2
  Merge2_Simulated515/1 -> Merge2_Simulated523/2
  Merge2_Simulated514/1 -> Merge2_Simulated522/2
  Merge2_Simulated513/1 -> Merge2_Simulated521/2
  Merge2_Simulated512/1 -> Merge2_Simulated520/2
  Merge2_Simulated518/1 -> Merge2_Simulated526/2
  Merge2_Simulated523/1 -> Merge2_Simulated531/2
  Merge2_Simulated244/1 -> Merge2_Simulated534/1
  Merge2_Simulated525/1 -> Merge2_Simulated533/2
  Merge2_Simulated227/1 -> Merge2_Simulated529/1
  Merge2_Simulated524/1 -> Merge2_Simulated532/2
  Merge2_Simulated520/1 -> Merge2_Simulated528/2
  Merge2_Simulated527/1 -> Merge2_Simulated535/2
  Merge2_Simulated254/1 -> Merge2_Simulated533/1
  Merge2_Simulated522/1 -> Merge2_Simulated530/2
  Merge2_Simulated192/1 -> Merge2_Simulated535/1
  Merge2_Simulated218/1 -> Merge2_Simulated530/1
  Merge2_Simulated235/1 -> Merge2_Simulated528/1
  Merge2_Simulated521/1 -> Merge2_Simulated529/2
  Merge2_Simulated200/1 -> Merge2_Simulated532/1
  Merge2_Simulated526/1 -> Merge2_Simulated534/2
  Merge2_Simulated209/1 -> Merge2_Simulated531/1
  Merge2_Simulated531/1 -> Merge2_Simulated539/2
  Merge2_Simulated308/1 -> Merge2_Simulated542/1
  Merge2_Simulated533/1 -> Merge2_Simulated541/2
  Merge2_Simulated291/1 -> Merge2_Simulated537/1
  Merge2_Simulated532/1 -> Merge2_Simulated540/2
  Merge2_Simulated528/1 -> Merge2_Simulated536/2
  Merge2_Simulated535/1 -> Merge2_Simulated543/2
  Merge2_Simulated318/1 -> Merge2_Simulated541/1
  Merge2_Simulated530/1 -> Merge2_Simulated538/2
  Merge2_Simulated256/1 -> Merge2_Simulated543/1
  Merge2_Simulated282/1 -> Merge2_Simulated538/1
  Merge2_Simulated299/1 -> Merge2_Simulated536/1
  Merge2_Simulated529/1 -> Merge2_Simulated537/2
  Merge2_Simulated264/1 -> Merge2_Simulated540/1
  Merge2_Simulated534/1 -> Merge2_Simulated542/2
  Merge2_Simulated273/1 -> Merge2_Simulated539/1
  Merge2_Simulated539/1 -> Merge2_Simulated547/2
  Merge2_Simulated372/1 -> Merge2_Simulated550/1
  Merge2_Simulated541/1 -> Merge2_Simulated549/2
  Merge2_Simulated355/1 -> Merge2_Simulated545/1
  Merge2_Simulated540/1 -> Merge2_Simulated548/2
  Merge2_Simulated536/1 -> Merge2_Simulated544/2
  Merge2_Simulated543/1 -> Merge2_Simulated551/2
  Merge2_Simulated382/1 -> Merge2_Simulated549/1
  Merge2_Simulated538/1 -> Merge2_Simulated546/2
  Merge2_Simulated320/1 -> Merge2_Simulated551/1
  Merge2_Simulated346/1 -> Merge2_Simulated546/1
  Merge2_Simulated363/1 -> Merge2_Simulated544/1
  Merge2_Simulated537/1 -> Merge2_Simulated545/2
  Merge2_Simulated328/1 -> Merge2_Simulated548/1
  Merge2_Simulated542/1 -> Merge2_Simulated550/2
  Merge2_Simulated337/1 -> Merge2_Simulated547/1
  Merge2_Simulated547/1 -> Merge2_Simulated555/2
  Merge2_Simulated436/1 -> Merge2_Simulated558/1
  Merge2_Simulated549/1 -> Merge2_Simulated557/2
  Merge2_Simulated419/1 -> Merge2_Simulated553/1
  Merge2_Simulated548/1 -> Merge2_Simulated556/2
  Merge2_Simulated544/1 -> Merge2_Simulated552/2
  Merge2_Simulated551/1 -> Merge2_Simulated559/2
  Merge2_Simulated446/1 -> Merge2_Simulated557/1
  Merge2_Simulated546/1 -> Merge2_Simulated554/2
  Merge2_Simulated384/1 -> Merge2_Simulated559/1
  Merge2_Simulated410/1 -> Merge2_Simulated554/1
  Merge2_Simulated427/1 -> Merge2_Simulated552/1
  Merge2_Simulated545/1 -> Merge2_Simulated553/2
  Merge2_Simulated392/1 -> Merge2_Simulated556/1
  Merge2_Simulated550/1 -> Merge2_Simulated558/2
  Merge2_Simulated401/1 -> Merge2_Simulated555/1
  Merge2_Simulated555/1 -> Merge2_Simulated563/2
  Merge2_Simulated500/1 -> Merge2_Simulated566/1
  Merge2_Simulated557/1 -> Merge2_Simulated565/2
  Merge2_Simulated483/1 -> Merge2_Simulated561/1
  Merge2_Simulated556/1 -> Merge2_Simulated564/2
  Merge2_Simulated552/1 -> Merge2_Simulated560/2
  Merge2_Simulated559/1 -> Merge2_Simulated567/2
  Merge2_Simulated510/1 -> Merge2_Simulated565/1
  Merge2_Simulated554/1 -> Merge2_Simulated562/2
  Merge2_Simulated448/1 -> Merge2_Simulated567/1
  Merge2_Simulated474/1 -> Merge2_Simulated562/1
  Merge2_Simulated491/1 -> Merge2_Simulated560/1
  Merge2_Simulated553/1 -> Merge2_Simulated561/2
  Merge2_Simulated456/1 -> Merge2_Simulated564/1
  Merge2_Simulated558/1 -> Merge2_Simulated566/2
  Merge2_Simulated465/1 -> Merge2_Simulated563/1
  Merge2_Simulated567/1 -> Row_7(1B)/1
  Merge2_Simulated565/1 -> Row_6(1B)/1
  Merge2_Simulated564/1 -> Row_5(1B)/1
  Merge2_Simulated566/1 -> Row_0(1B)/1
  Merge2_Simulated560/1 -> Row_1(1B)/1
  Merge2_Simulated561/1 -> Row_2(1B)/1
  Merge2_Simulated562/1 -> Row_3(1B)/1
  Merge2_Simulated563/1 -> Row_4(1B)/1
  Dec_8/8 -> Bitmap_Enable/1, Bitmap_Enable1/1, Bitmap_Enable2/1, Bitmap_Enable3/1, Bitmap_Enable4/1, Bitmap_Enable5/1, Bitmap_Enable6/1, Bitmap_Enable7/1
  Dec_8/7 -> Bitmap_Enable8/1, Bitmap_Enable9/1, Bitmap_Enable10/1, Bitmap_Enable11/1, Bitmap_Enable12/1, Bitmap_Enable13/1, Bitmap_Enable14/1, Bitmap_Enable15/1
  Dec_8/6 -> Bitmap_Enable16/1, Bitmap_Enable17/1, Bitmap_Enable18/1, Bitmap_Enable19/1, Bitmap_Enable20/1, Bitmap_Enable21/1, Bitmap_Enable22/1, Bitmap_Enable23/1
  Dec_8/5 -> Bitmap_Enable24/1, Bitmap_Enable25/1, Bitmap_Enable26/1, Bitmap_Enable27/1, Bitmap_Enable28/1, Bitmap_Enable29/1, Bitmap_Enable30/1, Bitmap_Enable31/1
  Dec_8/4 -> Bitmap_Enable32/1, Bitmap_Enable33/1, Bitmap_Enable34/1, Bitmap_Enable35/1, Bitmap_Enable36/1, Bitmap_Enable37/1, Bitmap_Enable38/1, Bitmap_Enable39/1
  Dec_8/3 -> Bitmap_Enable40/1, Bitmap_Enable41/1, Bitmap_Enable42/1, Bitmap_Enable43/1, Bitmap_Enable44/1, Bitmap_Enable45/1, Bitmap_Enable46/1, Bitmap_Enable47/1
  Dec_8/2 -> Bitmap_Enable48/1, Bitmap_Enable49/1, Bitmap_Enable50/1, Bitmap_Enable51/1, Bitmap_Enable52/1, Bitmap_Enable53/1, Bitmap_Enable54/1, Bitmap_Enable55/1
  Dec_8/1 -> Bitmap_Enable56/1, Bitmap_Enable57/1, Bitmap_Enable58/1, Bitmap_Enable59/1, Bitmap_Enable60/1, Bitmap_Enable61/1, Bitmap_Enable62/1, Bitmap_Enable63/1
  Align8/1 -> Bitmap_Enable15/2, Bitmap_Enable23/2, Bitmap_Enable31/2, Bitmap_Enable39/2, Bitmap_Enable47/2, Bitmap_Enable63/2, Bitmap_Enable55/2, Bitmap_Enable7/2
  Align8/2 -> Bitmap_Enable6/2, Bitmap_Enable14/2, Bitmap_Enable22/2, Bitmap_Enable30/2, Bitmap_Enable38/2, Bitmap_Enable46/2, Bitmap_Enable54/2, Bitmap_Enable62/2
  Align8/3 -> Bitmap_Enable5/2, Bitmap_Enable13/2, Bitmap_Enable21/2, Bitmap_Enable29/2, Bitmap_Enable37/2, Bitmap_Enable45/2, Bitmap_Enable53/2, Bitmap_Enable61/2
  Align8/4 -> Bitmap_Enable4/2, Bitmap_Enable12/2, Bitmap_Enable20/2, Bitmap_Enable28/2, Bitmap_Enable36/2, Bitmap_Enable44/2, Bitmap_Enable52/2, Bitmap_Enable60/2
  Align8/5 -> Bitmap_Enable3/2, Bitmap_Enable11/2, Bitmap_Enable19/2, Bitmap_Enable27/2, Bitmap_Enable35/2, Bitmap_Enable43/2, Bitmap_Enable51/2, Bitmap_Enable59/2
  Align8/6 -> Bitmap_Enable2/2, Bitmap_Enable10/2, Bitmap_Enable18/2, Bitmap_Enable26/2, Bitmap_Enable34/2, Bitmap_Enable42/2, Bitmap_Enable50/2, Bitmap_Enable58/2
  Align8/7 -> Bitmap_Enable1/2, Bitmap_Enable9/2, Bitmap_Enable17/2, Bitmap_Enable25/2, Bitmap_Enable33/2, Bitmap_Enable41/2, Bitmap_Enable49/2, Bitmap_Enable57/2
  Align8/8 -> Bitmap_Enable/2, Bitmap_Enable40/2, Bitmap_Enable48/2, Bitmap_Enable56/2, Bitmap_Enable32/2, Bitmap_Enable24/2, Bitmap_Enable16/2, Bitmap_Enable8/2
  Dec_1/8 -> Align8/1
  Dec_1/7 -> Align8/2
  Dec_1/6 -> Align8/3
  Dec_1/5 -> Align8/4
  Dec_1/4 -> Align8/5
  Dec_1/3 -> Align8/6
  Dec_1/2 -> Align8/7
  Dec_1/1 -> Align8/8
  OrdNum(1B)/1 -> Bus Selector1/1
  Bus Selector1/6 -> Dec_1/3  "<b00>"
  Bus Selector1/5 -> Dec_1/2  "<b01>"
  Bus Selector1/4 -> Dec_1/1  "<b02>"
  Bus Selector1/3 -> Dec_8/3  "<b03>"
  Bus Selector1/2 -> Dec_8/2  "<b04>"
  Bus Selector1/1 -> Dec_8/1  "<b05>"
